simulink model "SF006A_TEstimn"  (R2013b)
settings: Solver=FixedStepDiscrete  StartTime=0.0  StopTime=1  FixedStep=0.1  RelTol=1e-3
values from neighbouring files (symbols this model uses):
  ARCHGLBPRM_100MILLISEC_SEC_F32 = DataDict.Constant    [SF006A_TEstimn_DataDict.m]
  ARCHGLBPRM_2MILLISEC_SEC_F32 = DataDict.Constant    [SF006A_TEstimn_DataDict.m]
  TEstimnAmbPwrMplr = DataDict.Calibration    [SF006A_TEstimn_DataDict.m]
  TEstimnAmbTSca = DataDict.Calibration    [SF006A_TEstimn_DataDict.m]
  TEstimnAssiMechAmbMplr = DataDict.Calibration    [SF006A_TEstimn_DataDict.m]
  TEstimnAssiMechCorrLim = DataDict.Calibration    [SF006A_TEstimn_DataDict.m]
  TEstimnAssiMechDampgSca = DataDict.Calibration    [SF006A_TEstimn_DataDict.m]
  TEstimnAssiMechDftT = DataDict.Calibration    [SF006A_TEstimn_DataDict.m]
  TEstimnAssiMechLLFilCoeffA1 = DataDict.Calibration    [SF006A_TEstimn_DataDict.m]
  TEstimnAssiMechLLFilCoeffB0 = DataDict.Calibration    [SF006A_TEstimn_DataDict.m]
  TEstimnAssiMechLLFilCoeffB1 = DataDict.Calibration    [SF006A_TEstimn_DataDict.m]
  TEstimnAssiMechSlew = DataDict.Calibration    [SF006A_TEstimn_DataDict.m]
  TESTIMNASSIMECHTHILIM_DEGCGRD_F32 = DataDict.Constant    [SF006A_TEstimn_DataDict.m]
  TESTIMNASSIMECHTLOLIM_DEGCGRD_F32 = DataDict.Constant    [SF006A_TEstimn_DataDict.m]
  TEstimnCorrnTAssiMech = DataDict.Calibration    [SF006A_TEstimn_DataDict.m]
  TEstimnCorrnTCu = DataDict.Calibration    [SF006A_TEstimn_DataDict.m]
  TEstimnCorrnTMag = DataDict.Calibration    [SF006A_TEstimn_DataDict.m]
  TEstimnCorrnTSi = DataDict.Calibration    [SF006A_TEstimn_DataDict.m]
  TEstimnCuAmbMplr = DataDict.Calibration    [SF006A_TEstimn_DataDict.m]
  TEstimnCuCorrnLim = DataDict.Calibration    [SF006A_TEstimn_DataDict.m]
  TEstimnCuLLFilCoeffA1 = DataDict.Calibration    [SF006A_TEstimn_DataDict.m]
  TEstimnCuLLFilCoeffB0 = DataDict.Calibration    [SF006A_TEstimn_DataDict.m]
  TEstimnCuLLFilCoeffB1 = DataDict.Calibration    [SF006A_TEstimn_DataDict.m]
  TEstimnEngTSca = DataDict.Calibration    [SF006A_TEstimn_DataDict.m]
  TESTIMNFETTHILIM_DEGCGRD_F32 = DataDict.Constant    [SF006A_TEstimn_DataDict.m]
  TESTIMNFETTLOLIM_DEGCGRD_F32 = DataDict.Constant    [SF006A_TEstimn_DataDict.m]
  TEstimnMagAmbMplr = DataDict.Calibration    [SF006A_TEstimn_DataDict.m]
  TEstimnMagCorrnLim = DataDict.Calibration    [SF006A_TEstimn_DataDict.m]
  TEstimnMagLLFilCoeffA1 = DataDict.Calibration    [SF006A_TEstimn_DataDict.m]
  TEstimnMagLLFilCoeffB0 = DataDict.Calibration    [SF006A_TEstimn_DataDict.m]
  TEstimnMagLLFilCoeffB1 = DataDict.Calibration    [SF006A_TEstimn_DataDict.m]
  TESTIMNMAGTHILIM_DEGCGRD_F32 = DataDict.Constant    [SF006A_TEstimn_DataDict.m]
  TESTIMNMAGTLOLIM_DEGCGRD_F32 = DataDict.Constant    [SF006A_TEstimn_DataDict.m]
  TEstimnSiAmbMplr = DataDict.Calibration    [SF006A_TEstimn_DataDict.m]
  TEstimnSiCorrnLim = DataDict.Calibration    [SF006A_TEstimn_DataDict.m]
  TEstimnSiLLFilCoeffA1 = DataDict.Calibration    [SF006A_TEstimn_DataDict.m]
  TEstimnSiLLFilCoeffB0 = DataDict.Calibration    [SF006A_TEstimn_DataDict.m]
  TEstimnSiLLFilCoeffB1 = DataDict.Calibration    [SF006A_TEstimn_DataDict.m]
  TEstimnWghtAvrgTDi = DataDict.Calibration    [SF006A_TEstimn_DataDict.m]
  TESTIMNWIDGTHILIM_DEGCGRD_F32 = DataDict.Constant    [SF006A_TEstimn_DataDict.m]
  TESTIMNWIDGTLOLIM_DEGCGRD_F32 = DataDict.Constant    [SF006A_TEstimn_DataDict.m]
undefined symbols (not defined in the file or in its folder): sigbuilder_block
libraries: NxtrLim x13, Fil x8, simulink x2
(part 1 of 3)
settings Model: Creator=PallavG  LastModifiedBy=FZG88Y
settings DataIOCC: LimitDataPoints=off  SaveFormat=Structure  ReturnWorkspaceOutputs=on
settings OptimizationCC: BlockReduction=off  InlineParams=on  ZeroExternalMemoryAtStartup=off  ZeroInternalMemoryAtStartup=off  OptimizeModelRefInitCode=on  LifeSpan=1
settings DebuggingCC: SignalInfNanChecking=error  SignalRangeChecking=warning  UnderspecifiedInitializationDetection=Simplified  SolverPrmCheckMsg=error  InheritedTsInSrcMsg=error  DiscreteInheritContinuousMsg=error  SingleTaskRateTransMsg=error  TasksWithSamePriorityMsg=error  SigSpecEnsureSampleTimeMsg=error  CheckMatrixSingularityMsg=error  IntegerOverflowMsg=error  ParameterUnderflowMsg=error  ParameterPrecisionLossMsg=error  ParameterTunabilityLossMsg=error  FixptConstUnderflowMsg=warning  FixptConstOverflowMsg=warning  VectorMatrixConversionMsg=error  SignalLabelMismatchMsg=error  UnconnectedInputMsg=error  UnconnectedOutputMsg=error  UnconnectedLineMsg=error  SFcnCompatibilityMsg=error  UniqueDataStoreMsg=warning  BusObjectLabelMismatch=error  RootOutportRequireBusObject=error  AssertControl=DisableAll  ModelReferenceIOMsg=error  ModelReferenceVersionMismatchMessage=warning  ModelReferenceIOMismatchMessage=error  ModelReferenceCSMismatchMessage=warning  ModelReferenceDataLoggingMessage=error  StateNameClashWarn=warning  StrictBusMsg=ErrorOnBusTreatedAsVector  NonBusSignalsTreatedAsBus=error  SFUnexpectedBacktrackingDiag=error  SFInvalidInputDataAccessInChartInitDiag=error  SFNoUnconditionalDefaultTransitionDiag=error  SFTransitionOutsideNaturalParentDiag=error  SFUnconditionalTransitionShadowingDiag=error  SFUndirectedBroadcastEventsDiag=error
settings ModelReferenceCC: ModelReferenceNumInstancesAllowed=Single
settings RTWCC: SystemTargetFile=autosar.tlc  GenCodeOnly=on  TemplateMakefile=ert_default_tmf  Description=AUTOSAR  GenerateReport=on  ProcessScript=autosar_make_rtw_hook  LaunchReport=on
settings CodeAppCC: GenerateComments=off  IgnoreCustomStorageClasses=off  CustomSymbolStrType=$N$R$M  CustomSymbolStrBlkIO=$N$M  SimulinkBlockComments=off
settings STFCustomTargetCC: ParMdlRefBuildCompliant=on  CompOptLevelCompliant=on  IncludeMdlTerminateFcn=off  CombineOutputUpdateFcns=on  SuppressErrorStatus=on  ERTFirstTimeCompliant=on  ERTCustomFileBanners=on  SupportNonFinite=off  SupportComplex=off  SupportContinuousTime=off  SupportNonInlinedSFcns=off  MATLABClassNameForMDSCustomization=Simulink.SoftwareTarget.ERTCustomization  AutosarCompliant=on  GRTInterface=off  SystemTargetFile=autosar.tlc
settings ERTTargetCC: CodeReplacementLibrary=ANSI_C  ConcurrentExecutionCompliant=off  IncludeMdlTerminateFcn=off  SuppressErrorStatus=on  SupportNonFinite=off  SupportComplex=off  ModelStepFunctionPrototypeControlCompliant=off  CPPClassGenCompliant=off  AutosarCompliant=on  InlinedParameterPlacement=NonHierarchical  ERTCustomFileTemplate=example_file_process.tlc  EnableUserReplacementTypes=on

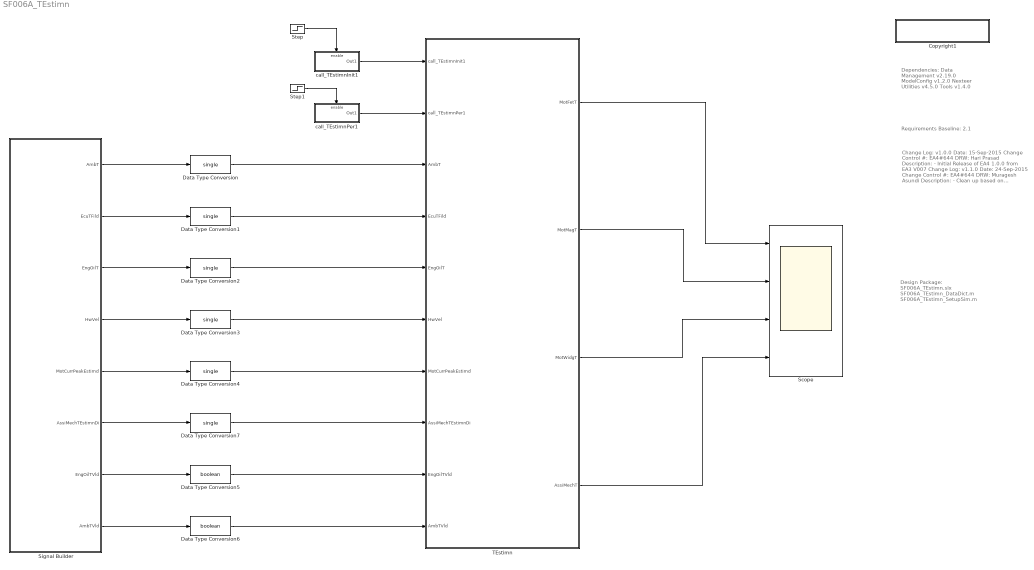
== system SF006A_TEstimn ==
  note: Requirements Baseline: 2.1
  note: Design Package:
      | SF006A_TEstimn.slx
      | SF006A_TEstimn_DataDict.m
      | SF006A_TEstimn_SetupSim.m
  note: Change Log:  v1.0.0
      | Date: 15-Sep-2015
      | Change Control #: EA4#644
      | DRW:  Hari Prasad
      | Description:
      | - Initial Release of EA4 1.0.0 from EA3 V007
      |
      | Change Log:  v1.1.0
      | Date: 24-Sep-2015
      | Change Control #: EA4#644
      | DRW:  Muragesh Asundi
      | Description:
      | - Clean up based on comments from SW team
  note: Dependencies:
      |    Data Management v2.19.0
      |    ModelConfig v1.2.0
      |    Nexteer Utilities v4.5.0
      |    Tools v1.4.0
  Copyright1 : Subsystem  Description=|  RequirementInfo={} %GIDa_31a5e494_f362_4315_ad68_df9135c8582b  mask(Copyright Information){none=on}
      | Copyright info block.                                               
      |                                                                     
      | Place copyright information at the top of every subsystem in design.
      mask prompts: none "No parameters"
      mask help: Place copyright information at the top of every subsystem in design.
      mask Display:
      | NxtrConf = 'Nexteer Confidential';
      | 
      | sys = bdroot; %handle for the current model ("system")
      | first = get_param(sys,'Created');
      | if(isempty(first))
      |     first = datestr(now,'yyyy');
      | else
      |     first = first(end-3:end);  %year is last four digits
      | end
      | 
      | last = get_param(sys,'LastModifiedDate');
      | if isempty(last)
      |     last = datestr(now,'yyyy');
      | else
      |     last = last(end-3:end);
      | end
      | 
      | if strcmp(first,last)
      |     fprintf('%s\nCopyright  %s Nexteer',NxtrConf,first);
      | else
      |     fprintf('%s\n%s%s-%s Nexteer',NxtrConf,char(169),first,last);
      | end
  Data Type Conversion{,1..4,7} (6 alike) : DataTypeConversion  OutDataTypeStr=single
  Data Type Conversion5 : DataTypeConversion  OutDataTypeStr=boolean
  Data Type Conversion6 : DataTypeConversion  OutDataTypeStr=boolean
  Scope : Scope  NumInputPorts=4
      settings: YMin=-5~-5~-5~-5  YMax=5~5~5~5
  Signal Builder : Subsystem  Tag=STV Subsys  LoadFcn=sigbuilder_block('load');  StartFcn=sigbuilder_block('start');  StopFcn=sigbuilder_block('stop');  ClipboardFcn=sigbuilder_block('clipboard');  mask(Sigbuilder block){}
      mask help: Simulink:masks:SigbuilderBlock_MD
      mask init:
      | if ~strcmp(get_param(bdroot(gcbh),'SimulationStatus'),'stopped') tuvar = sigbuilder_block('maskInit'); end
      settings: CopyFcn=sigbuilder_block('copy');  DeleteFcn=sigbuilder_block('delete');  ModelCloseFcn=sigbuilder_block('modelClose');  PreSaveFcn=sigbuilder_block('preSave');  PauseFcn=sigbuilder_block('pause');  ContinueFcn=sigbuilder_block('continue');  NameChangeFcn=sigbuilder_block('namechange');  OpenFcn=sigbuilder_block('open',[84 66 786.75 394.5 ]);  CloseFcn=sigbuilder_block('close');
      mask Display: plot(0, 0, 100, 100,[2, 2, 32, 32, 2], [68, 8, 8, 68, 68],[32, 2], [38, 38], [32, 19, 2],[53, 60, 44], [32, 17, 17, 2],[16, 16, 31, 31]);txt = getActiveGroup(gcbh);text(2, 100, txt,'verticalAlignment', 'top');
  Step : Step  Time=.001  Before=1  After=0  SampleTime=0
  Step1 : Step  Time=0.001  SampleTime=0.1
  TEstimn : Subsystem  RequirementInfo={'linktype_rmi_doors' '0000a528 (/E-STEER Core/SubSystem Specifications/Application Functions/SF006A Temperature Estimation)' '#SF006A_113' 'true' 'REQ: SF006A_113' '' } %GIDa_45cdad98_892c_499b_8f4d_04ff41f4306a
  call_TEstimnInit1 : Subsystem  TreatAsAtomicUnit=on
  call_TEstimnPer1 : Subsystem  TreatAsAtomicUnit=on
  wires:
  TEstimn/4(AssiMechT) -> Scope/4
  TEstimn/3(MotWidgT) -> Scope/3
  TEstimn/2(MotMagT) -> Scope/2
  TEstimn/1(MotFetT) -> Scope/1
  Data Type Conversion/1 -> TEstimn/3(AmbT)
  Data Type Conversion1/1 -> TEstimn/4(EcuTFild)
  Data Type Conversion2/1 -> TEstimn/5(EngOilT)
  Data Type Conversion3/1 -> TEstimn/6(HwVel)
  Data Type Conversion4/1 -> TEstimn/7(MotCurrPeakEstimd)
  Data Type Conversion7/1 -> TEstimn/8(AssiMechTEstimnDi)
  Signal Builder/7(EngOilTVld) -> Data Type Conversion5/1
  Signal Builder/2(EcuTFild) -> Data Type Conversion1/1
  Signal Builder/5(MotCurrPeakEstimd) -> Data Type Conversion4/1
  Signal Builder/3(EngOilT) -> Data Type Conversion2/1
  Signal Builder/6(AssiMechTEstimnDi) -> Data Type Conversion7/1
  Signal Builder/4(HwVel) -> Data Type Conversion3/1
  Signal Builder/1(AmbT) -> Data Type Conversion/1
  Data Type Conversion6/1 -> TEstimn/10(AmbTVld)
  Data Type Conversion5/1 -> TEstimn/9(EngOilTVld)
  Signal Builder/8(AmbTVld) -> Data Type Conversion6/1
  Step/1 -> call_TEstimnInit1/Enable
  call_TEstimnInit1/1(Out1) -> TEstimn/1(call_TEstimnInit1)
  Step1/1 -> call_TEstimnPer1/Enable
  call_TEstimnPer1/1(Out1) -> TEstimn/2(call_TEstimnPer1)

== system SF006A_TEstimn/Copyright1 ==

== system SF006A_TEstimn/Signal Builder ==
  Demux : Demux  Tag=STV Demux  Outputs=8
  FromWs : FromWorkspace  Tag=STV FromWs  VariableName=tuvar  SampleTime=0
      SigBuilderData=|
      | common.afterFinalStr = 'Extrapolate'
      | common.sampleTime = 0
      | dataSet(1).timeRange = [0 0.11]
      | dataSet(1).name = 'TestCase1'
      | dataSet(2).timeRange = [0 0.11]
      | dataSet(2).name = 'TestCase2'
      | dataSet(3).timeRange = [0 0.11]
      | dataSet(3).name = 'TestCase3'
      | dataSet(4).timeRange = [0 0.11]
      | dataSet(4).name = 'TestCase4'
      | dataSet(5).timeRange = [0 0.11]
      | dataSet(5).name = 'TestCase5'
      | dataSet(6).timeRange = [0 0.11]
      | dataSet(6).name = 'TestCase6'
      | sbobj.Name = 'Signal Builder'
      | sbobj.Groups(1).Name = 'TestCase1'
      | sbobj.Groups(1).Signals(1).Name = 'AmbT'
      | sbobj.Groups(1).Signals(1).XData = [0 0.002 0.004 0.006 0.008 0.01 0.012 0.014 0.016 0.018 0.02 0.022 0.024 0.026 0.028 0.03 0.032 0.034 0.036 0.038 0.04 0.042 0.044 0.046 0.048 0.05 0.052 0.054 0.056 0.058 0.06 0.062 0.064 0.066 0.068 0.07 0.072 0.074 0.076 0.078 0.08 0.082 0.084 0.086 0.088 0.09 0.092 0.094 0.096 0.098 0.1 0.102 0.104 0.106 0.108 0.11]
      | sbobj.Groups(1).Signals(1).YData = [0 0 0 0 0 0 0 0 0 0 0 0 0 0 0 0 0 0 0 0 0 0 0 0 0 0 0 0 0 0 0 0 0 0 0 0 0 0 0 0 0 0 0 0 0 0 0 0 0 0 0 0 0 0 0 0]
      | sbobj.Groups(1).Signals(2).Name = 'EcuTFild'
      | sbobj.Groups(1).Signals(2).XData = [0 0.002 0.004 0.006 0.008 0.01 0.012 0.014 0.016 0.018 0.02 0.022 0.024 0.026 0.028 0.03 0.032 0.034 0.036 0.038 0.04 0.042 0.044 0.046 0.048 0.05 0.052 0.054 0.056 0.058 0.06 0.062 0.064 0.066 0.068 0.07 0.072 0.074 0.076 0.078 0.08 0.082 0.084 0.086 0.088 0.09 0.092 0.094 0.096 0.098 0.1 0.102 0.104 0.106 0.108 0.11]
      | sbobj.Groups(1).Signals(2).YData = [50 50 23 -10 50 -3 50 50 -50 50 50 -25 50 50 -18 50 50 100 50 34 50 67 50 50 50 123 50 50 50 88 50 111 50 50 50 92 50 50 146 50 50 50 50 50 50 50 50 50 50 50 50 50 50 50 50 50]
      | sbobj.Groups(1).Signals(3).Name = 'EngOilT'
      | sbobj.Groups(1).Signals(3).XData = [0 0.002 0.004 0.006 0.008 0.01 0.012 0.014 0.016 0.018 0.02 0.022 0.024 0.026 0.028 0.03 0.032 0.034 0.036 0.038 0.04 0.042 0.044 0.046 0.048 0.05 0.052 0.054 0.056 0.058 0.06 0.062 0.064 0.066 0.068 0.07 0.072 0.074 0.076 0.078 0.08 0.082 0.084 0.086 0.088 0.09 0.092 0.094 0.096 0.098 0.1 0.102 0.104 0.106 0.108 0.11]
      | sbobj.Groups(1).Signals(3).YData = [5 5 5 5 5 5 5 5 5 5 5 5 5 5 -5 5 5 5 5 -20 5 5 5 5 -10 5 5 5 5 5 5 5 5 5 5 5 5 5 5 5 5 5 5 5 5 5 5 5 5 5 5 5 5 5 5 5]
      | sbobj.Groups(1).Signals(4).Name = 'HwVel'
      | sbobj.Groups(1).Signals(4).XData = [0 0.002 0.004 0.006 0.008 0.01 0.012 0.014 0.016 0.018 0.02 0.022 0.024 0.026 0.028 0.03 0.032 0.034 0.036 0.038 0.04 0.042 0.044 0.046 0.048 0.05 0.052 0.054 0.056 0.058 0.06 0.062 0.064 0.066 0.068 0.07 0.072 0.074 0.076 0.078 0.08 0.082 0.084 0.086 0.088 0.09 0.092 0.094 0.096 0.098 0.1 0.102 0.104 0.106 0.108 0.11]
      | sbobj.Groups(1).Signals(4).YData = [3 3 3 3 3 3 3 3 3 3 3 3 3 3 3 3 3 3 3 3 3 3 3 3 3 3 3 3 3 3 3 3 3 3 3 3 3 3 3 3 3 3 3 3 3 3 3 3 3 3 3 3 3 3 3 3]
      | sbobj.Groups(1).Signals(5).Name = 'MotCurrPeakEstimd'
      | sbobj.Groups(1).Signals(5).XData = [0 0.002 0.004 0.006 0.008 0.01 0.012 0.014 0.016 0.018 0.02 0.022 0.024 0.026 0.028 0.03 0.032 0.034 0.036 0.038 0.04 0.042 0.044 0.046 0.048 0.05 0.052 0.054 0.056 0.058 0.06 0.062 0.064 0.066 0.068 0.07 0.072 0.074 0.076 0.078 0.08 0.082 0.084 0.086 0.088 0.09 0.092 0.094 0.096 0.098 0.1 0.102 0.104 0.106 0.108 0.11]
      | sbobj.Groups(1).Signals(5).YData = [5 5 5 5 5 5 5 5 5 5 5 5 5 5 5 5 5 5 5 5 5 5 5 5 5 5 5 5 5 5 5 5 5 5 5 5 5 5 5 5 5 5 5 5 5 5 5 5 5 5 5 5 5 5 5 5]
      | sbobj.Groups(1).Signals(6).Name = 'AssiMechTEstimnDi'
      | sbobj.Groups(1).Signals(6).XData = [0 0.002 0.004 0.006 0.008 0.01 0.012 0.014 0.016 0.018 0.02 0.022 0.024 0.026 0.028 0.03 0.032 0.034 0.036 0.038 0.04 0.042 0.044 0.046 0.048 0.05 0.052 0.054 0.056 0.058 0.06 0.062 0.064 0.066 0.068 0.07 0.072 0.074 0.076 0.078 0.08 0.082 0.084 0.086 0.088 0.09 0.092 0.094 0.096 0.098 0.1 0.102 0.104 0.106 0.108 0.11]
      | sbobj.Groups(1).Signals(6).YData = [0 0 0 0 0 0 0 0 0 0 0 0 0 0 0 0 0 0 0 0 0 0 0 0 0 0 0 0 0 0 0 0 0 0 0 0 0 0 0 0 0 0 0 0 0 0 0 0 0 0 0 0 0 0 0 0]
      | sbobj.Groups(1).Signals(7).Name = 'EngOilTVld'
      | sbobj.Groups(1).Signals(7).XData = [0 0.002 0.004 0.006 0.008 0.01 0.012 0.014 0.016 0.018 0.02 0.022 0.024 0.026 0.028 0.03 0.032 0.034 0.036 0.038 0.04 0.042 0.044 0.046 0.048 0.05 0.052 0.054 0.056 0.058 0.06 0.062 0.064 0.066 0.068 0.07 0.072 0.074 0.076 0.078 0.08 0.082 0.084 0.086 0.088 0.09 0.092 0.094 0.096 0.098 0.1 0.102 0.104 0.106 0.108 0.11]
      | sbobj.Groups(1).Signals(7).YData = [1 1 1 1 1 1 1 1 1 1 1 1 1 1 1 1 1 1 1 1 1 1 1 1 1 1 1 1 1 1 1 1 1 1 1 1 1 1 1 1 1 1 1 1 1 1 1 1 1 1 1 1 1 1 1 1]
      | sbobj.Groups(1).Signals(8).Name = 'AmbTVld'
      | sbobj.Groups(1).Signals(8).XData = [0 0.002 0.004 0.006 0.008 0.01 0.012 0.014 0.016 0.018 0.02 0.022 0.024 0.026 0.028 0.03 0.032 0.034 0.036 0.038 0.04 0.042 0.044 0.046 0.048 0.05 0.052 0.054 0.056 0.058 0.06 0.062 0.064 0.066 0.068 0.07 0.072 0.074 0.076 0.078 0.08 0.082 0.084 0.086 0.088 0.09 0.092 0.094 0.096 0.098 0.1 0.102 0.104 0.106 0.108 0.11]
      | sbobj.Groups(1).Signals(8).YData = [1 1 1 1 1 1 1 1 1 1 1 1 1 1 1 1 1 1 1 1 1 1 1 1 1 1 1 1 1 1 1 1 1 1 1 1 1 1 1 1 1 1 1 1 1 1 1 1 1 1 1 1 1 1 1 1]
      | sbobj.Groups(1).TimeRange = [0 0.11]
      | sbobj.Groups(2).Name = 'TestCase2'
      | sbobj.Groups(2).Signals(1).Name = 'AmbT'
      | sbobj.Groups(2).Signals(1).XData = [0 0.002 0.004 0.006 0.008 0.01 0.012 0.014 0.016 0.018 0.02 0.022 0.024 0.026 0.028 0.03 0.032 0.034 0.036 0.038 0.04 0.042 0.044 0.046 0.048 0.05 0.052 0.054 0.056 0.058 0.06 0.062 0.064 0.066 0.068 0.07 0.072 0.074 0.076 0.078 0.08 0.082 0.084 0.086 0.088 0.09 0.092 0.094 0.096 0.098 0.1 0.102 0.104 0.106 0.108 0.11]
      | sbobj.Groups(2).Signals(1).YData = [0 0 0 0 0 0 0 0 0 0 0 0 0 0 0 0 0 0 0 0 0 0 0 0 0 0 0 0 0 0 0 0 0 0 0 0 0 0 0 0 0 0 0 0 0 0 0 0 0 0 0 0 0 0 0 0]
      | sbobj.Groups(2).Signals(2).Name = 'EcuTFild'
      | sbobj.Groups(2).Signals(2).XData = [0 0.002 0.004 0.006 0.008 0.01 0.012 0.014 0.016 0.018 0.02 0.022 0.024 0.026 0.028 0.03 0.032 0.034 0.036 0.038 0.04 0.042 0.044 0.046 0.048 0.05 0.052 0.054 0.056 0.058 0.06 0.062 0.064 0.066 0.068 0.07 0.072 0.074 0.076 0.078 0.08 0.082 0.084 0.086 0.088 0.09 0.092 0.094 0.096 0.098 0.1 0.102 0.104 0.106 0.108 0.11]
      | sbobj.Groups(2).Signals(2).YData = [50 50 50 50 50 50 50 50 50 50 50 50 50 50 50 50 50 50 50 50 50 50 50 50 50 50 50 50 50 50 50 50 50 50 50 50 50 50 50 50 50 50 50 50 50 50 50 50 50 50 50 50 50 50 50 50]
      | sbobj.Groups(2).Signals(3).Name = 'EngOilT'
      | sbobj.Groups(2).Signals(3).XData = [0 0.002 0.004 0.006 0.008 0.01 0.012 0.014 0.016 0.018 0.02 0.022 0.024 0.026 0.028 0.03 0.032 0.034 0.036 0.038 0.04 0.042 0.044 0.046 0.048 0.05 0.052 0.054 0.056 0.058 0.06 0.062 0.064 0.066 0.068 0.07 0.072 0.074 0.076 0.078 0.08 0.082 0.084 0.086 0.088 0.09 0.092 0.094 0.096 0.098 0.1 0.102 0.104 0.106 0.108 0.11]
      | sbobj.Groups(2).Signals(3).YData = [-20 5 -11 5 5 -2 5 22 5 5 -8 5 98 5 -5 5 -50 5 5 -20 5 5 100 5 -10 5 59 5 5 67 5 5 5 90 5 -1 5 88 5 5 1 5 5 5 23 5 56 5 5 5 5 123 5 0 5 102]
      | sbobj.Groups(2).Signals(4).Name = 'HwVel'
      | sbobj.Groups(2).Signals(4).XData = [0 0.002 0.004 0.006 0.008 0.01 0.012 0.014 0.016 0.018 0.02 0.022 0.024 0.026 0.028 0.03 0.032 0.034 0.036 0.038 0.04 0.042 0.044 0.046 0.048 0.05 0.052 0.054 0.056 0.058 0.06 0.062 0.064 0.066 0.068 0.07 0.072 0.074 0.076 0.078 0.08 0.082 0.084 0.086 0.088 0.09 0.092 0.094 0.096 0.098 0.1 0.102 0.104 0.106 0.108 0.11]
      | sbobj.Groups(2).Signals(4).YData = [3 3 3 3 3 3 3 3 3 3 3 3 3 3 3 3 3 3 3 3 3 3 3 3 3 3 3 3 3 3 3 3 3 3 3 3 3 3 3 3 3 3 3 3 3 3 3 3 3 3 3 3 3 3 3 3]
      | sbobj.Groups(2).Signals(5).Name = 'MotCurrPeakEstimd'
      | sbobj.Groups(2).Signals(5).XData = [0 0.002 0.004 0.006 0.008 0.01 0.012 0.014 0.016 0.018 0.02 0.022 0.024 0.026 0.028 0.03 0.032 0.034 0.036 0.038 0.04 0.042 0.044 0.046 0.048 0.05 0.052 0.054 0.056 0.058 0.06 0.062 0.064 0.066 0.068 0.07 0.072 0.074 0.076 0.078 0.08 0.082 0.084 0.086 0.088 0.09 0.092 0.094 0.096 0.098 0.1 0.102 0.104 0.106 0.108 0.11]
      | sbobj.Groups(2).Signals(5).YData = [5 5 5 5 5 5 5 5 5 5 5 5 5 5 5 5 5 5 5 5 5 5 5 5 5 5 5 5 5 5 5 5 5 5 5 5 5 5 5 5 5 5 5 5 5 5 5 5 5 5 5 5 5 5 5 5]
      | sbobj.Groups(2).Signals(6).Name = 'AssiMechTEstimnDi'
      | sbobj.Groups(2).Signals(6).XData = [0 0.002 0.004 0.006 0.008 0.01 0.012 0.014 0.016 0.018 0.02 0.022 0.024 0.026 0.028 0.03 0.032 0.034 0.036 0.038 0.04 0.042 0.044 0.046 0.048 0.05 0.052 0.054 0.056 0.058 0.06 0.062 0.064 0.066 0.068 0.07 0.072 0.074 0.076 0.078 0.08 0.082 0.084 0.086 0.088 0.09 0.092 0.094 0.096 0.098 0.1 0.102 0.104 0.106 0.108 0.11]
      | sbobj.Groups(2).Signals(6).YData = [0 0 0 0 0 0 0 0 0 0 0 0 0 0 0 0 0 0 0 0 0 0 0 0 0 0 0 0 0 0 0 0 0 0 0 0 0 0 0 0 0 0 0 0 0 0 0 0 0 0 0 0 0 0 0 0]
      | sbobj.Groups(2).Signals(7).Name = 'EngOilTVld'
      | sbobj.Groups(2).Signals(7).XData = [0 0.002 0.004 0.006 0.008 0.01 0.012 0.014 0.016 0.018 0.02 0.022 0.024 0.026 0.028 0.03 0.032 0.034 0.036 0.038 0.04 0.042 0.044 0.046 0.048 0.05 0.052 0.054 0.056 0.058 0.06 0.062 0.064 0.066 0.068 0.07 0.072 0.074 0.076 0.078 0.08 0.082 0.084 0.086 0.088 0.09 0.092 0.094 0.096 0.098 0.1 0.102 0.104 0.106 0.108 0.11]
      | sbobj.Groups(2).Signals(7).YData = [1 1 1 1 1 1 1 1 1 1 1 1 1 1 1 1 1 1 1 1 1 1 1 1 1 1 1 1 1 1 1 1 1 1 1 1 1 1 1 1 1 1 1 1 1 1 1 1 1 1 1 1 1 1 1 1]
      | sbobj.Groups(2).Signals(8).Name = 'AmbTVld'
      | sbobj.Groups(2).Signals(8).XData = [0 0.002 0.004 0.006 0.008 0.01 0.012 0.014 0.016 0.018 0.02 0.022 0.024 0.026 0.028 0.03 0.032 0.034 0.036 0.038 0.04 0.042 0.044 0.046 0.048 0.05 0.052 0.054 0.056 0.058 0.06 0.062 0.064 0.066 0.068 0.07 0.072 0.074 0.076 0.078 0.08 0.082 0.084 0.086 0.088 0.09 0.092 0.094 0.096 0.098 0.1 0.102 0.104 0.106 0.108 0.11]
      | sbobj.Groups(2).Signals(8).YData = [1 1 1 1 1 1 1 1 1 1 1 1 1 1 1 1 1 1 1 1 1 1 1 1 1 1 1 1 1 1 1 1 1 1 1 1 1 1 1 1 1 1 1 1 1 1 1 1 1 1 1 1 1 1 1 1]
      | sbobj.Groups(2).TimeRange = [0 0.11]
      | sbobj.Groups(3).Name = 'TestCase3'
      | sbobj.Groups(3).Signals(1).Name = 'AmbT'
      | sbobj.Groups(3).Signals(1).XData = [0 0.002 0.004 0.006 0.008 0.01 0.012 0.014 0.016 0.018 0.02 0.022 0.024 0.026 0.028 0.03 0.032 0.034 0.036 0.038 0.04 0.042 0.044 0.046 0.048 0.05 0.052 0.054 0.056 0.058 0.06 0.062 0.064 0.066 0.068 0.07 0.072 0.074 0.076 0.078 0.08 0.082 0.084 0.086 0.088 0.09 0.092 0.094 0.096 0.098 0.1 0.102 0.104 0.106 0.108 0.11]
      | sbobj.Groups(3).Signals(1).YData = [0 0 0 0 0 0 0 0 0 0 0 0 0 0 0 0 0 0 0 0 0 0 0 0 0 0 0 0 0 0 0 0 0 0 0 0 0 0 0 0 0 0 0 0 0 0 0 0 0 0 0 0 0 0 0 0]
      | sbobj.Groups(3).Signals(2).Name = 'EcuTFild'
      | sbobj.Groups(3).Signals(2).XData = [0 0.002 0.004 0.006 0.008 0.01 0.012 0.014 0.016 0.018 0.02 0.022 0.024 0.026 0.028 0.03 0.032 0.034 0.036 0.038 0.04 0.042 0.044 0.046 0.048 0.05 0.052 0.054 0.056 0.058 0.06 0.062 0.064 0.066 0.068 0.07 0.072 0.074 0.076 0.078 0.08 0.082 0.084 0.086 0.088 0.09 0.092 0.094 0.096 0.098 0.1 0.102 0.104 0.106 0.108 0.11]
      | sbobj.Groups(3).Signals(2).YData = [50 50 50 50 50 50 50 50 50 50 50 50 50 50 50 50 50 50 50 50 50 50 50 50 50 50 50 50 50 50 50 50 50 50 50 50 50 50 50 50 50 50 50 50 50 50 50 50 50 50 50 50 50 50 50 50]
      | sbobj.Groups(3).Signals(3).Name = 'EngOilT'
      | sbobj.Groups(3).Signals(3).XData = [0 0.002 0.004 0.006 0.008 0.01 0.012 0.014 0.016 0.018 0.02 0.022 0.024 0.026 0.028 0.03 0.032 0.034 0.036 0.038 0.04 0.042 0.044 0.046 0.048 0.05 0.052 0.054 0.056 0.058 0.06 0.062 0.064 0.066 0.068 0.07 0.072 0.074 0.076 0.078 0.08 0.082 0.084 0.086 0.088 0.09 0.092 0.094 0.096 0.098 0.1 0.102 0.104 0.106 0.108 0.11]
      | sbobj.Groups(3).Signals(3).YData = [5 5 5 5 5 5 5 5 5 5 5 5 5 5 -5 5 5 5 5 -20 5 5 5 5 -10 5 5 5 5 5 5 5 5 5 5 5 5 5 5 5 5 5 5 5 5 5 5 5 5 5 5 5 5 5 5 5]
      | sbobj.Groups(3).Signals(4).Name = 'HwVel'
      | sbobj.Groups(3).Signals(4).XData = [0 0.002 0.004 0.006 0.008 0.01 0.012 0.014 0.016 0.018 0.02 0.022 0.024 0.026 0.028 0.03 0.032 0.034 0.036 0.038 0.04 0.042 0.044 0.046 0.048 0.05 0.052 0.054 0.056 0.058 0.06 0.062 0.064 0.066 0.068 0.07 0.072 0.074 0.076 0.078 0.08 0.082 0.084 0.086 0.088 0.09 0.092 0.094 0.096 0.098 0.1 0.102 0.104 0.106 0.108 0.11]
      | sbobj.Groups(3).Signals(4).YData = [-42 -40 -30 32 3 3 3 33 3 40 3 3 3 3 23 3 3 0 3 3 3 3 29 3 3 10 3 3 3 -1 3 3 3 3 -3 3 3 3 3 18 3 3 -5 3 11 3 3 -10 3 3 9 3 3 40 21 42]
      | sbobj.Groups(3).Signals(5).Name = 'MotCurrPeakEstimd'
      | sbobj.Groups(3).Signals(5).XData = [0 0.002 0.004 0.006 0.008 0.01 0.012 0.014 0.016 0.018 0.02 0.022 0.024 0.026 0.028 0.03 0.032 0.034 0.036 0.038 0.04 0.042 0.044 0.046 0.048 0.05 0.052 0.054 0.056 0.058 0.06 0.062 0.064 0.066 0.068 0.07 0.072 0.074 0.076 0.078 0.08 0.082 0.084 0.086 0.088 0.09 0.092 0.094 0.096 0.098 0.1 0.102 0.104 0.106 0.108 0.11]
      | sbobj.Groups(3).Signals(5).YData = [5 5 5 5 5 5 5 5 5 5 5 5 5 5 5 5 5 5 5 5 5 5 5 5 5 5 5 5 5 5 5 5 5 5 5 5 5 5 5 5 5 5 5 5 5 5 5 5 5 5 5 5 5 5 5 5]
      | sbobj.Groups(3).Signals(6).Name = 'AssiMechTEstimnDi'
      | sbobj.Groups(3).Signals(6).XData = [0 0.002 0.004 0.006 0.008 0.01 0.012 0.014 0.016 0.018 0.02 0.022 0.024 0.026 0.028 0.03 0.032 0.034 0.036 0.038 0.04 0.042 0.044 0.046 0.048 0.05 0.052 0.054 0.056 0.058 0.06 0.062 0.064 0.066 0.068 0.07 0.072 0.074 0.076 0.078 0.08 0.082 0.084 0.086 0.088 0.09 0.092 0.094 0.096 0.098 0.1 0.102 0.104 0.106 0.108 0.11]
      | sbobj.Groups(3).Signals(6).YData = [0 0 0 0 0 0 0 0 0 0 0 0 0 0 0 0 0 0 0 0 0 0 0 0 0 0 0 0 0 0 0 0 0 0 0 0 0 0 0 0 0 0 0 0 0 0 0 0 0 0 0 0 0 0 0 0]
      | sbobj.Groups(3).Signals(7).Name = 'EngOilTVld'
      | sbobj.Groups(3).Signals(7).XData = [0 0.002 0.004 0.006 0.008 0.01 0.012 0.014 0.016 0.018 0.02 0.022 0.024 0.026 0.028 0.03 0.032 0.034 0.036 0.038 0.04 0.042 0.044 0.046 0.048 0.05 0.052 0.054 0.056 0.058 0.06 0.062 0.064 0.066 0.068 0.07 0.072 0.074 0.076 0.078 0.08 0.082 0.084 0.086 0.088 0.09 0.092 0.094 0.096 0.098 0.1 0.102 0.104 0.106 0.108 0.11]
      | sbobj.Groups(3).Signals(7).YData = [1 1 1 1 1 1 1 1 1 1 1 1 1 1 1 1 1 1 1 1 1 1 1 1 1 1 1 1 1 1 1 1 1 1 1 1 1 1 1 1 1 1 1 1 1 1 1 1 1 1 1 1 1 1 1 1]
      | sbobj.Groups(3).Signals(8).Name = 'AmbTVld'
      | sbobj.Groups(3).Signals(8).XData = [0 0.002 0.004 0.006 0.008 0.01 0.012 0.014 0.016 0.018 0.02 0.022 0.024 0.026 0.028 0.03 0.032 0.034 0.036 0.038 0.04 0.042 0.044 0.046 0.048 0.05 0.052 0.054 0.056 0.058 0.06 0.062 0.064 0.066 0.068 0.07 0.072 0.074 0.076 0.078 0.08 0.082 0.084 0.086 0.088 0.09 0.092 0.094 0.096 0.098 0.1 0.102 0.104 0.106 0.108 0.11]
      | sbobj.Groups(3).Signals(8).YData = [1 1 1 1 1 1 1 1 1 1 1 1 1 1 1 1 1 1 1 1 1 1 1 1 1 1 1 1 1 1 1 1 1 1 1 1 1 1 1 1 1 1 1 1 1 1 1 1 1 1 1 1 1 1 1 1]
      | sbobj.Groups(3).TimeRange = [0 0.11]
      | sbobj.Groups(4).Name = 'TestCase4'
      | sbobj.Groups(4).Signals(1).Name = 'AmbT'
      | sbobj.Groups(4).Signals(1).XData = [0 0.002 0.004 0.006 0.008 0.01 0.012 0.014 0.016 0.018 0.02 0.022 0.024 0.026 0.028 0.03 0.032 0.034 0.036 0.038 0.04 0.042 0.044 0.046 0.048 0.05 0.052 0.054 0.056 0.058 0.06 0.062 0.064 0.066 0.068 0.07 0.072 0.074 0.076 0.078 0.08 0.082 0.084 0.086 0.088 0.09 0.092 0.094 0.096 0.098 0.1 0.102 0.104 0.106 0.108 0.11]
      | sbobj.Groups(4).Signals(1).YData = [0 0 0 0 0 0 0 0 0 0 0 0 0 0 0 0 0 0 0 0 0 0 0 0 0 0 0 0 0 0 0 0 0 0 0 0 0 0 0 0 0 0 0 0 0 0 0 0 0 0 0 0 0 0 0 0]
      | sbobj.Groups(4).Signals(2).Name = 'EcuTFild'
      | sbobj.Groups(4).Signals(2).XData = [0 0.002 0.004 0.006 0.008 0.01 0.012 0.014 0.016 0.018 0.02 0.022 0.024 0.026 0.028 0.03 0.032 0.034 0.036 0.038 0.04 0.042 0.044 0.046 0.048 0.05 0.052 0.054 0.056 0.058 0.06 0.062 0.064 0.066 0.068 0.07 0.072 0.074 0.076 0.078 0.08 0.082 0.084 0.086 0.088 0.09 0.092 0.094 0.096 0.098 0.1 0.102 0.104 0.106 0.108 0.11]
      | sbobj.Groups(4).Signals(2).YData = [50 50 50 50 50 50 50 50 50 50 50 50 50 50 50 50 50 50 50 50 50 50 50 50 50 50 50 50 50 50 50 50 50 50 50 50 50 50 50 50 50 50 50 50 50 50 50 50 50 50 50 50 50 50 50 50]
      | sbobj.Groups(4).Signals(3).Name = 'EngOilT'
      | sbobj.Groups(4).Signals(3).XData = [0 0.002 0.004 0.006 0.008 0.01 0.012 0.014 0.016 0.018 0.02 0.022 0.024 0.026 0.028 0.03 0.032 0.034 0.036 0.038 0.04 0.042 0.044 0.046 0.048 0.05 0.052 0.054 0.056 0.058 0.06 0.062 0.064 0.066 0.068 0.07 0.072 0.074 0.076 0.078 0.08 0.082 0.084 0.086 0.088 0.09 0.092 0.094 0.096 0.098 0.1 0.102 0.104 0.106 0.108 0.11]
      | sbobj.Groups(4).Signals(3).YData = [5 5 5 5 5 5 5 5 5 5 5 5 5 5 -5 5 5 5 5 -20 5 5 5 5 -10 5 5 5 5 5 5 5 5 5 5 5 5 5 5 5 5 5 5 5 5 5 5 5 5 5 5 5 5 5 5 5]
      | sbobj.Groups(4).Signals(4).Name = 'HwVel'
      | sbobj.Groups(4).Signals(4).XData = [0 0.002 0.004 0.006 0.008 0.01 0.012 0.014 0.016 0.018 0.02 0.022 0.024 0.026 0.028 0.03 0.032 0.034 0.036 0.038 0.04 0.042 0.044 0.046 0.048 0.05 0.052 0.054 0.056 0.058 0.06 0.062 0.064 0.066 0.068 0.07 0.072 0.074 0.076 0.078 0.08 0.082 0.084 0.086 0.088 0.09 0.092 0.094 0.096 0.098 0.1 0.102 0.104 0.106 0.108 0.11]
      | sbobj.Groups(4).Signals(4).YData = [3 3 3 3 3 3 3 3 3 3 3 3 3 3 3 3 3 3 3 3 3 3 3 3 3 3 3 3 3 3 3 3 3 3 3 3 3 3 3 3 3 3 3 3 3 3 3 3 3 3 3 3 3 3 3 3]
      | sbobj.Groups(4).Signals(5).Name = 'MotCurrPeakEstimd'
      | sbobj.Groups(4).Signals(5).XData = [0 0.002 0.004 0.006 0.008 0.01 0.012 0.014 0.016 0.018 0.02 0.022 0.024 0.026 0.028 0.03 0.032 0.034 0.036 0.038 0.04 0.042 0.044 0.046 0.048 0.05 0.052 0.054 0.056 0.058 0.06 0.062 0.064 0.066 0.068 0.07 0.072 0.074 0.076 0.078 0.08 0.082 0.084 0.086 0.088 0.09 0.092 0.094 0.096 0.098 0.1 0.102 0.104 0.106 0.108 0.11]
      | sbobj.Groups(4).Signals(5).YData = [100 5 5 30000 5 5 5 24000 5 5 456 5 5 21 5 5 3245 5 22 5 5 0 5 5 999 5 5 5 1919 5 5 5 34 5 5 5657 5 5 10000 5 5 9879 5 5 62500 5 5 5 66 5 5 0 5 9 5 100]
      | sbobj.Groups(4).Signals(6).Name = 'AssiMechTEstimnDi'
      | sbobj.Groups(4).Signals(6).XData = [0 0.002 0.004 0.006 0.008 0.01 0.012 0.014 0.016 0.018 0.02 0.022 0.024 0.026 0.028 0.03 0.032 0.034 0.036 0.038 0.04 0.042 0.044 0.046 0.048 0.05 0.052 0.054 0.056 0.058 0.06 0.062 0.064 0.066 0.068 0.07 0.072 0.074 0.076 0.078 0.08 0.082 0.084 0.086 0.088 0.09 0.092 0.094 0.096 0.098 0.1 0.102 0.104 0.106 0.108 0.11]
      | sbobj.Groups(4).Signals(6).YData = [0 0 0 0 0 0 0 0 0 0 0 0 0 0 0 0 0 0 0 0 0 0 0 0 0 0 0 0 0 0 0 0 0 0 0 0 0 0 0 0 0 0 0 0 0 0 0 0 0 0 0 0 0 0 0 0]
      | sbobj.Groups(4).Signals(7).Name = 'EngOilTVld'
      | sbobj.Groups(4).Signals(7).XData = [0 0.002 0.004 0.006 0.008 0.01 0.012 0.014 0.016 0.018 0.02 0.022 0.024 0.026 0.028 0.03 0.032 0.034 0.036 0.038 0.04 0.042 0.044 0.046 0.048 0.05 0.052 0.054 0.056 0.058 0.06 0.062 0.064 0.066 0.068 0.07 0.072 0.074 0.076 0.078 0.08 0.082 0.084 0.086 0.088 0.09 0.092 0.094 0.096 0.098 0.1 0.102 0.104 0.106 0.108 0.11]
      | sbobj.Groups(4).Signals(7).YData = [1 1 1 1 1 1 1 1 1 1 1 1 1 1 1 1 1 1 1 1 1 1 1 1 1 1 1 1 1 1 1 1 1 1 1 1 1 1 1 1 1 1 1 1 1 1 1 1 1 1 1 1 1 1 1 1]
      | sbobj.Groups(4).Signals(8).Name = 'AmbTVld'
      | sbobj.Groups(4).Signals(8).XData = [0 0.002 0.004 0.006 0.008 0.01 0.012 0.014 0.016 0.018 0.02 0.022 0.024 0.026 0.028 0.03 0.032 0.034 0.036 0.038 0.04 0.042 0.044 0.046 0.048 0.05 0.052 0.054 0.056 0.058 0.06 0.062 0.064 0.066 0.068 0.07 0.072 0.074 0.076 0.078 0.08 0.082 0.084 0.086 0.088 0.09 0.092 0.094 0.096 0.098 0.1 0.102 0.104 0.106 0.108 0.11]
      | sbobj.Groups(4).Signals(8).YData = [1 1 1 1 1 1 1 1 1 1 1 1 1 1 1 1 1 1 1 1 1 1 1 1 1 1 1 1 1 1 1 1 1 1 1 1 1 1 1 1 1 1 1 1 1 1 1 1 1 1 1 1 1 1 1 1]
      | sbobj.Groups(4).TimeRange = [0 0.11]
      | sbobj.Groups(5).Name = 'TestCase5'
      | sbobj.Groups(5).Signals(1).Name = 'AmbT'
      | sbobj.Groups(5).Signals(1).XData = [0 0.002 0.004 0.006 0.008 0.01 0.012 0.014 0.016 0.018 0.02 0.022 0.024 0.026 0.028 0.03 0.032 0.034 0.036 0.038 0.04 0.042 0.044 0.046 0.048 0.05 0.052 0.054 0.056 0.058 0.06 0.062 0.064 0.066 0.068 0.07 0.072 0.074 0.076 0.078 0.08 0.082 0.084 0.086 0.088 0.09 0.092 0.094 0.096 0.098 0.1 0.102 0.104 0.106 0.108 0.11]
      | sbobj.Groups(5).Signals(1).YData = [0 0 0 0 0 0 0 0 0 0 0 0 0 0 0 0 0 0 0 0 0 0 0 0 0 0 0 0 0 0 0 0 0 0 0 0 0 0 0 0 0 0 0 0 0 0 0 0 0 0 0 0 0 0 0 0]
      | sbobj.Groups(5).Signals(2).Name = 'EcuTFild'
      | sbobj.Groups(5).Signals(2).XData = [0 0.002 0.004 0.006 0.008 0.01 0.012 0.014 0.016 0.018 0.02 0.022 0.024 0.026 0.028 0.03 0.032 0.034 0.036 0.038 0.04 0.042 0.044 0.046 0.048 0.05 0.052 0.054 0.056 0.058 0.06 0.062 0.064 0.066 0.068 0.07 0.072 0.074 0.076 0.078 0.08 0.082 0.084 0.086 0.088 0.09 0.092 0.094 0.096 0.098 0.1 0.102 0.104 0.106 0.108 0.11]
      | sbobj.Groups(5).Signals(2).YData = [50 50 50 50 50 50 50 50 50 50 50 50 50 50 50 50 50 50 50 50 50 50 50 50 50 50 50 50 50 50 50 50 50 50 50 50 50 50 50 50 50 50 50 50 50 50 50 50 50 50 50 50 50 50 50 50]
      | sbobj.Groups(5).Signals(3).Name = 'EngOilT'
      | sbobj.Groups(5).Signals(3).XData = [0 0.002 0.004 0.006 0.008 0.01 0.012 0.014 0.016 0.018 0.02 0.022 0.024 0.026 0.028 0.03 0.032 0.034 0.036 0.038 0.04 0.042 0.044 0.046 0.048 0.05 0.052 0.054 0.056 0.058 0.06 0.062 0.064 0.066 0.068 0.07 0.072 0.074 0.076 0.078 0.08 0.082 0.084 0.086 0.088 0.09 0.092 0.094 0.096 0.098 0.1 0.102 0.104 0.106 0.108 0.11]
      | sbobj.Groups(5).Signals(3).YData = [5 5 5 5 5 5 5 5 5 5 5 5 5 5 -5 5 5 5 5 -20 5 5 5 5 -10 5 5 5 5 5 5 5 5 5 5 5 5 5 5 5 5 5 5 5 5 5 5 5 5 5 5 5 5 5 5 5]
      | sbobj.Groups(5).Signals(4).Name = 'HwVel'
      | sbobj.Groups(5).Signals(4).XData = [0 0.002 0.004 0.006 0.008 0.01 0.012 0.014 0.016 0.018 0.02 0.022 0.024 0.026 0.028 0.03 0.032 0.034 0.036 0.038 0.04 0.042 0.044 0.046 0.048 0.05 0.052 0.054 0.056 0.058 0.06 0.062 0.064 0.066 0.068 0.07 0.072 0.074 0.076 0.078 0.08 0.082 0.084 0.086 0.088 0.09 0.092 0.094 0.096 0.098 0.1 0.102 0.104 0.106 0.108 0.11]
      | sbobj.Groups(5).Signals(4).YData = [3 3 3 3 3 3 3 3 3 3 3 3 3 3 3 3 3 3 3 3 3 3 3 3 3 3 3 3 3 3 3 3 3 3 3 3 3 3 3 3 3 3 3 3 3 3 3 3 3 3 3 3 3 3 3 3]
      | sbobj.Groups(5).Signals(5).Name = 'MotCurrPeakEstimd'
      | sbobj.Groups(5).Signals(5).XData = [0 0.002 0.004 0.006 0.008 0.01 0.012 0.014 0.016 0.018 0.02 0.022 0.024 0.026 0.028 0.03 0.032 0.034 0.036 0.038 0.04 0.042 0.044 0.046 0.048 0.05 0.052 0.054 0.056 0.058 0.06 0.062 0.064 0.066 0.068 0.07 0.072 0.074 0.076 0.078 0.08 0.082 0.084 0.086 0.088 0.09 0.092 0.094 0.096 0.098 0.1 0.102 0.104 0.106 0.108 0.11]
      | sbobj.Groups(5).Signals(5).YData = [5 5 5 5 5 5 5 5 5 5 5 5 5 5 5 5 5 5 5 5 5 5 5 5 5 5 5 5 5 5 5 5 5 5 5 5 5 5 5 5 5 5 5 5 5 5 5 5 5 5 5 5 5 5 5 5]
      | sbobj.Groups(5).Signals(6).Name = 'AssiMechTEstimnDi'
      | sbobj.Groups(5).Signals(6).XData = [0 0.002 0.004 0.006 0.008 0.01 0.012 0.014 0.016 0.018 0.02 0.022 0.024 0.026 0.028 0.03 0.032 0.034 0.036 0.038 0.04 0.042 0.044 0.046 0.048 0.05 0.052 0.054 0.056 0.058 0.06 0.062 0.064 0.066 0.068 0.07 0.072 0.074 0.076 0.078 0.08 0.082 0.084 0.086 0.088 0.09 0.092 0.094 0.096 0.098 0.1 0.102 0.104 0.106 0.108 0.11]
      | sbobj.Groups(5).Signals(6).YData = [1 0 1 0 1 0 0 0 0 1 0 0 0 0 1 0 0 0 1 0 0 0 1 0 0 0 0 1 0 0 1 1 0 0 1 0 0 0 0 0 1 0 1 1 1 1 1 1 0 0 0 0 0 0 1 1]
      | sbobj.Groups(5).Signals(7).Name = 'EngOilTVld'
      | sbobj.Groups(5).Signals(7).XData = [0 0.002 0.004 0.006 0.008 0.01 0.012 0.014 0.016 0.018 0.02 0.022 0.024 0.026 0.028 0.03 0.032 0.034 0.036 0.038 0.04 0.042 0.044 0.046 0.048 0.05 0.052 0.054 0.056 0.058 0.06 0.062 0.064 0.066 0.068 0.07 0.072 0.074 0.076 0.078 0.08 0.082 0.084 0.086 0.088 0.09 0.092 0.094 0.096 0.098 0.1 0.102 0.104 0.106 0.108 0.11]
      | sbobj.Groups(5).Signals(7).YData = [1 1 1 1 1 1 1 1 1 1 1 1 1 1 1 1 1 1 1 1 1 1 1 1 1 1 1 1 1 1 1 1 1 1 1 1 1 1 1 1 1 1 1 1 1 1 1 1 1 1 1 1 1 1 1 1]
      | sbobj.Groups(5).Signals(8).Name = 'AmbTVld'
      | sbobj.Groups(5).Signals(8).XData = [0 0.002 0.004 0.006 0.008 0.01 0.012 0.014 0.016 0.018 0.02 0.022 0.024 0.026 0.028 0.03 0.032 0.034 0.036 0.038 0.04 0.042 0.044 0.046 0.048 0.05 0.052 0.054 0.056 0.058 0.06 0.062 0.064 0.066 0.068 0.07 0.072 0.074 0.076 0.078 0.08 0.082 0.084 0.086 0.088 0.09 0.092 0.094 0.096 0.098 0.1 0.102 0.104 0.106 0.108 0.11]
      | sbobj.Groups(5).Signals(8).YData = [1 1 1 1 1 1 1 1 1 1 1 1 1 1 1 1 1 1 1 1 1 1 1 1 1 1 1 1 1 1 1 1 1 1 1 1 1 1 1 1 1 1 1 1 1 1 1 1 1 1 1 1 1 1 1 1]
      | sbobj.Groups(5).TimeRange = [0 0.11]
      | sbobj.Groups(6).Name = 'TestCase6'
      | sbobj.Groups(6).Signals(1).Name = 'AmbT'
      | sbobj.Groups(6).Signals(1).XData = [0 0.002 0.004 0.006 0.008 0.01 0.012 0.014 0.016 0.018 0.02 0.022 0.024 0.026 0.028 0.03 0.032 0.034 0.036 0.038 0.04 0.042 0.044 0.046 0.048 0.05 0.052 0.054 0.056 0.058 0.06 0.062 0.064 0.066 0.068 0.07 0.072 0.074 0.076 0.078 0.08 0.082 0.084 0.086 0.088 0.09 0.092 0.094 0.096 0.098 0.1 0.102 0.104 0.106 0.108 0.11]
      | sbobj.Groups(6).Signals(1).YData = [0 0 0 0 0 0 0 0 0 0 0 0 0 0 0 0 0 0 0 0 0 0 0 0 0 0 0 0 0 0 0 0 0 0 0 0 0 0 0 0 0 0 0 0 0 0 0 0 0 0 0 0 0 0 0 0]
      | sbobj.Groups(6).Signals(2).Name = 'EcuTFild'
      | sbobj.Groups(6).Signals(2).XData = [0 0.002 0.004 0.006 0.008 0.01 0.012 0.014 0.016 0.018 0.02 0.022 0.024 0.026 0.028 0.03 0.032 0.034 0.036 0.038 0.04 0.042 0.044 0.046 0.048 0.05 0.052 0.054 0.056 0.058 0.06 0.062 0.064 0.066 0.068 0.07 0.072 0.074 0.076 0.078 0.08 0.082 0.084 0.086 0.088 0.09 0.092 0.094 0.096 0.098 0.1 0.102 0.104 0.106 0.108 0.11]
      | sbobj.Groups(6).Signals(2).YData = [50 50 50 50 50 50 50 50 50 50 50 50 50 50 50 50 50 50 50 50 50 50 50 50 50 50 50 50 50 50 50 50 50 50 50 50 50 50 50 50 50 50 50 50 50 50 50 50 50 50 50 50 50 50 50 50]
      | sbobj.Groups(6).Signals(3).Name = 'EngOilT'
      | sbobj.Groups(6).Signals(3).XData = [0 0.002 0.004 0.006 0.008 0.01 0.012 0.014 0.016 0.018 0.02 0.022 0.024 0.026 0.028 0.03 0.032 0.034 0.036 0.038 0.04 0.042 0.044 0.046 0.048 0.05 0.052 0.054 0.056 0.058 0.06 0.062 0.064 0.066 0.068 0.07 0.072 0.074 0.076 0.078 0.08 0.082 0.084 0.086 0.088 0.09 0.092 0.094 0.096 0.098 0.1 0.102 0.104 0.106 0.108 0.11]
      | sbobj.Groups(6).Signals(3).YData = [5 5 5 5 5 5 5 5 5 5 5 5 5 5 -5 5 5 5 5 -20 5 5 5 5 -10 5 5 5 5 5 5 5 5 5 5 5 5 5 5 5 5 5 5 5 5 5 5 5 5 5 5 5 5 5 5 5]
      | sbobj.Groups(6).Signals(4).Name = 'HwVel'
      | sbobj.Groups(6).Signals(4).XData = [0 0.002 0.004 0.006 0.008 0.01 0.012 0.014 0.016 0.018 0.02 0.022 0.024 0.026 0.028 0.03 0.032 0.034 0.036 0.038 0.04 0.042 0.044 0.046 0.048 0.05 0.052 0.054 0.056 0.058 0.06 0.062 0.064 0.066 0.068 0.07 0.072 0.074 0.076 0.078 0.08 0.082 0.084 0.086 0.088 0.09 0.092 0.094 0.096 0.098 0.1 0.102 0.104 0.106 0.108 0.11]
      | sbobj.Groups(6).Signals(4).YData = [3 3 3 3 3 3 3 3 3 3 3 3 3 3 3 3 3 3 3 3 3 3 3 3 3 3 3 3 3 3 3 3 3 3 3 3 3 3 3 3 3 3 3 3 3 3 3 3 3 3 3 3 3 3 3 3]
      | sbobj.Groups(6).Signals(5).Name = 'MotCurrPeakEstimd'
      | sbobj.Groups(6).Signals(5).XData = [0 0.002 0.004 0.006 0.008 0.01 0.012 0.014 0.016 0.018 0.02 0.022 0.024 0.026 0.028 0.03 0.032 0.034 0.036 0.038 0.04 0.042 0.044 0.046 0.048 0.05 0.052 0.054 0.056 0.058 0.06 0.062 0.064 0.066 0.068 0.07 0.072 0.074 0.076 0.078 0.08 0.082 0.084 0.086 0.088 0.09 0.092 0.094 0.096 0.098 0.1 0.102 0.104 0.106 0.108 0.11]
      | sbobj.Groups(6).Signals(5).YData = [5 5 5 5 5 5 5 5 5 5 5 5 5 5 5 5 5 5 5 5 5 5 5 5 5 5 5 5 5 5 5 5 5 5 5 5 5 5 5 5 5 5 5 5 5 5 5 5 5 5 5 5 5 5 5 5]
      | sbobj.Groups(6).Signals(6).Name = 'AssiMechTEstimnDi'
      | sbobj.Groups(6).Signals(6).XData = [0 0.002 0.004 0.006 0.008 0.01 0.012 0.014 0.016 0.018 0.02 0.022 0.024 0.026 0.028 0.03 0.032 0.034 0.036 0.038 0.04 0.042 0.044 0.046 0.048 0.05 0.052 0.054 0.056 0.058 0.06 0.062 0.064 0.066 0.068 0.07 0.072 0.074 0.076 0.078 0.08 0.082 0.084 0.086 0.088 0.09 0.092 0.094 0.096 0.098 0.1 0.102 0.104 0.106 0.108 0.11]
      | sbobj.Groups(6).Signals(6).YData = [1 0 1 0 1 0 0 0 0 1 0 0 0 0 1 0 0 0 1 0 0 1 1 1 0 0 0 1 0 0 1 1 1 1 1 1 1 1 0 0 1 0 1 1 1 1 1 1 0 0 0 0 1 1 1 1]
      | sbobj.Groups(6).Signals(7).Name = 'EngOilTVld'
      | sbobj.Groups(6).Signals(7).XData = [0 0.002 0.004 0.006 0.008 0.01 0.012 0.014 0.016 0.018 0.02 0.022 0.024 0.026 0.028 0.03 0.032 0.034 0.036 0.038 0.04 0.042 0.044 0.046 0.048 0.05 0.052 0.054 0.056 0.058 0.06 0.062 0.064 0.066 0.068 0.07 0.072 0.074 0.076 0.078 0.08 0.082 0.084 0.086 0.088 0.09 0.092 0.094 0.096 0.098 0.1 0.102 0.104 0.106 0.108 0.11]
      | sbobj.Groups(6).Signals(7).YData = [1 1 1 1 1 1 1 1 1 1 1 1 1 1 1 1 1 1 1 1 1 1 1 1 1 1 1 1 1 1 1 1 1 1 1 1 1 1 1 1 1 1 1 1 1 1 1 1 1 1 1 1 1 1 1 1]
      | sbobj.Groups(6).Signals(8).Name = 'AmbTVld'
      | sbobj.Groups(6).Signals(8).XData = [0 0.002 0.004 0.006 0.008 0.01 0.012 0.014 0.016 0.018 0.02 0.022 0.024 0.026 0.028 0.03 0.032 0.034 0.036 0.038 0.04 0.042 0.044 0.046 0.048 0.05 0.052 0.054 0.056 0.058 0.06 0.062 0.064 0.066 0.068 0.07 0.072 0.074 0.076 0.078 0.08 0.082 0.084 0.086 0.088 0.09 0.092 0.094 0.096 0.098 0.1 0.102 0.104 0.106 0.108 0.11]
      | sbobj.Groups(6).Signals(8).YData = [0 0 0 0 0 0 0 0 0 0 0 0 0 0 0 0 0 0 0 0 0 0 0 0 0 0 0 0 0 0 0 0 0 0 0 0 0 0 0 0 0 0 0 0 0 0 0 0 0 0 0 0 0 0 0 0]
      | sbobj.Groups(6).TimeRange = [0 0.11]
  AmbT : Outport
  EcuTFild : Outport  Tag=STV Outport  Port=2
  EngOilT : Outport  Tag=STV Outport  Port=3
  HwVel : Outport  Tag=STV Outport  Port=4
  MotCurrPeakEstimd : Outport  Tag=STV Outport  Port=5
  AssiMechTEstimnDi : Outport  Tag=STV Outport  Port=6
  EngOilTVld : Outport  Tag=STV Outport  Port=7
  AmbTVld : Outport  Tag=STV Outport  Port=8
  wires:
  Demux/1 -> AmbT/1
  FromWs/1 -> Demux/1
  Demux/2 -> EcuTFild/1
  Demux/3 -> EngOilT/1
  Demux/4 -> HwVel/1
  Demux/5 -> MotCurrPeakEstimd/1
  Demux/6 -> AssiMechTEstimnDi/1
  Demux/7 -> EngOilTVld/1
  Demux/8 -> AmbTVld/1

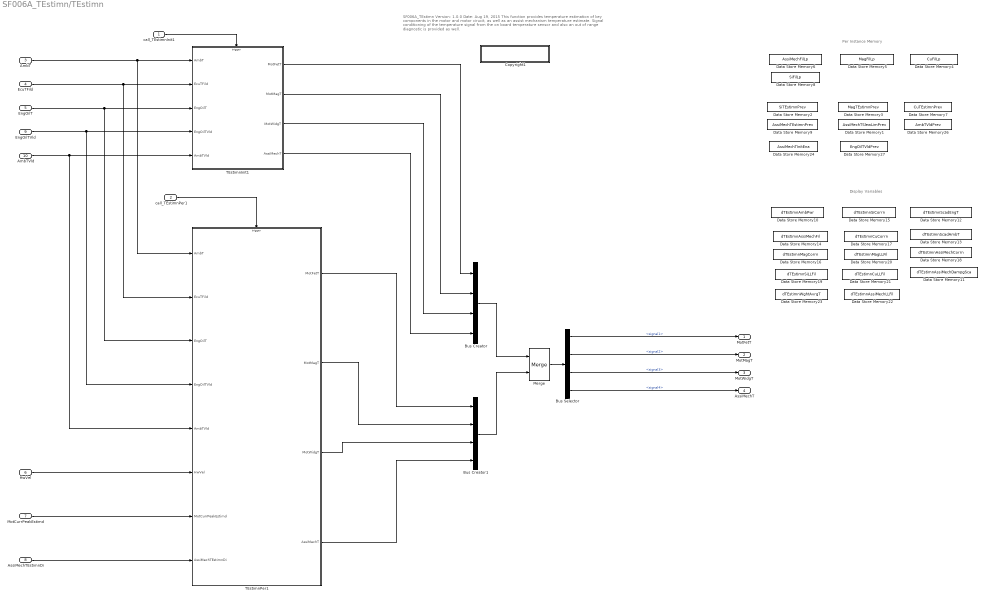
== system SF006A_TEstimn/TEstimn ==
  note: Per Instance Memory
  note: Display Variables
  note: SF006A_TEstimn       Version: 1.0.0                                                      Date:  Aug 19, 2015
      |
      | This function provides temperature estimation of key components in the motor and motor cirucit, as well as an assist mechanism temperature estimate.
      |  Signal conditioning of the temperature signal from the on board temperature sensor and also an out of range diagnostic is provided as well.
  call_TEstimnInit1 : Inport
  call_TEstimnPer1 : Inport  Port=2
  AmbT : Inport  RequirementInfo={'linktype_rmi_doors' '0000a528 (/E-STEER Core/SubSystem Specifications/Application Functions/SF006A Temperature Estimation)' '#SF006A_36' 'true' 'REQ: SF006A_36' '' } %GIDa_5d6b064d_6b6f_4541_a887_c0efbe9c0c94  Port=3
  EcuTFild : Inport  RequirementInfo={'linktype_rmi_doors' '0000a528 (/E-STEER Core/SubSystem Specifications/Application Functions/SF006A Temperature Estimation)' '#SF006A_169' 'true' 'REQ: SF006A_169' '' } %GIDa_7589b720_6e4c_4e94_96af_7b6fe1e4d0db  Port=4
  EngOilT : Inport  RequirementInfo={'linktype_rmi_doors' '0000a528 (/E-STEER Core/SubSystem Specifications/Application Functions/SF006A Temperature Estimation)' '#SF006A_35' 'true' 'REQ: SF006A_35' '' } %GIDa_5c47e2cc_0424_4f9b_9e07_6d85924c893e  Port=5
  HwVel : Inport  RequirementInfo={'linktype_rmi_doors' '0000a528 (/E-STEER Core/SubSystem Specifications/Application Functions/SF006A Temperature Estimation)' '#SF006A_33' 'true' 'REQ: SF006A_33' '' } %GIDa_66961606_1485_4273_a568_ee274f5fd10b  Port=6
  MotCurrPeakEstimd : Inport  RequirementInfo={'linktype_rmi_doors' '0000a528 (/E-STEER Core/SubSystem Specifications/Application Functions/SF006A Temperature Estimation)' '#SF006A_34' 'true' 'REQ: SF006A_34' '' } %GIDa_9ffd1575_018e_4c04_9a89_090695dc7784  Port=7
  AssiMechTEstimnDi : Inport  RequirementInfo={'linktype_rmi_doors' '0000a528 (/E-STEER Core/SubSystem Specifications/Application Functions/SF006A Temperature Estimation)' '#SF006A_39' 'true' 'REQ: SF006A_39' '' } %GIDa_64c39ffe_14e6_405a_a806_1cae4ba36277  Port=8
  EngOilTVld : Inport  RequirementInfo={'linktype_rmi_doors' '0000a528 (/E-STEER Core/SubSystem Specifications/Application Functions/SF006A Temperature Estimation)' '#SF006A_37' 'true' 'REQ: SF006A_37' '' } %GIDa_7d7a5cea_4edb_4765_a58d_84344722e689  Port=9
  AmbTVld : Inport  RequirementInfo={'linktype_rmi_doors' '0000a528 (/E-STEER Core/SubSystem Specifications/Application Functions/SF006A Temperature Estimation)' '#SF006A_37' 'true' 'REQ: SF006A_37' '' } %GIDa_744f25b6_7177_4752_87bb_5589619ff46a  Port=10
  Bus Creator : BusCreator
  Bus Creator1 : BusCreator
  Bus Selector : BusSelector  OutputSignals=signal1,signal2,signal3,signal4
  Copyright1 : Subsystem  Description=|  RequirementInfo={} %GIDa_40b2bef5_baed_40e1_9760_ec08ea904b84  mask(Copyright Information){none=on}
      | Copyright info block.                                               
      |                                                                     
      | Place copyright information at the top of every subsystem in design.
      mask prompts: none "No parameters"
      mask help: Place copyright information at the top of every subsystem in design.
      mask Display:
      | NxtrConf = 'Nexteer Confidential';
      | 
      | sys = bdroot; %handle for the current model ("system")
      | first = get_param(sys,'Created');
      | if(isempty(first))
      |     first = datestr(now,'yyyy');
      | else
      |     first = first(end-3:end);  %year is last four digits
      | end
      | 
      | last = get_param(sys,'LastModifiedDate');
      | if isempty(last)
      |     last = datestr(now,'yyyy');
      | else
      |     last = last(end-3:end);
      | end
      | 
      | if strcmp(first,last)
      |     fprintf('%s\nCopyright  %s Nexteer',NxtrConf,first);
      | else
      |     fprintf('%s\n%s%s-%s Nexteer',NxtrConf,char(169),first,last);
      | end
  Data Store Memory1 : DataStoreMemory  DataStoreName=AssiMechTSlewLimPrev  StateMustResolveToSignalObject=on
      settings: LockScale=on
  Data Store Memory10 : DataStoreMemory  DataStoreName=dTEstimnAmbPwr  StateMustResolveToSignalObject=on
  Data Store Memory11 : DataStoreMemory  DataStoreName=dTEstimnAssiMechDampgSca  StateMustResolveToSignalObject=on
  Data Store Memory12 : DataStoreMemory  DataStoreName=dTEstimnScadEngT  StateMustResolveToSignalObject=on
  Data Store Memory13 : DataStoreMemory  DataStoreName=dTEstimnScadAmbT  StateMustResolveToSignalObject=on
  Data Store Memory14 : DataStoreMemory  DataStoreName=dTEstimnAssiMechFil  StateMustResolveToSignalObject=on
  Data Store Memory15 : DataStoreMemory  DataStoreName=dTEstimnSiCorrn  StateMustResolveToSignalObject=on
  Data Store Memory16 : DataStoreMemory  DataStoreName=dTEstimnMagCorrn  StateMustResolveToSignalObject=on
  Data Store Memory17 : DataStoreMemory  DataStoreName=dTEstimnCuCorrn  StateMustResolveToSignalObject=on
  Data Store Memory18 : DataStoreMemory  DataStoreName=dTEstimnAssiMechCorrn  StateMustResolveToSignalObject=on
  Data Store Memory19 : DataStoreMemory  DataStoreName=dTEstimnSiLLFil  StateMustResolveToSignalObject=on
  Data Store Memory2 : DataStoreMemory  DataStoreName=SiTEstimnPrev  StateMustResolveToSignalObject=on
  Data Store Memory20 : DataStoreMemory  DataStoreName=dTEstimnMagLLFil  StateMustResolveToSignalObject=on
  Data Store Memory21 : DataStoreMemory  DataStoreName=dTEstimnCuLLFil  StateMustResolveToSignalObject=on
  Data Store Memory22 : DataStoreMemory  DataStoreName=dTEstimnAssiMechLLFil  StateMustResolveToSignalObject=on
  Data Store Memory23 : DataStoreMemory  DataStoreName=dTEstimnWghtAvrgT  StateMustResolveToSignalObject=on
  Data Store Memory24 : DataStoreMemory  DataStoreName=AssiMechTInitEna  StateMustResolveToSignalObject=on
      settings: LockScale=on
  Data Store Memory26 : DataStoreMemory  DataStoreName=AmbTVldPrev  StateMustResolveToSignalObject=on
  Data Store Memory27 : DataStoreMemory  DataStoreName=EngOilTVldPrev  StateMustResolveToSignalObject=on
  Data Store Memory3 : DataStoreMemory  DataStoreName=MagTEstimnPrev  StateMustResolveToSignalObject=on
  Data Store Memory4 : DataStoreMemory  DataStoreName=CuFilLp  InitialValue=struct('FilSt',single(0),'FilGain',single(0))  OutDataTypeStr=Bus: FilLpRec1  StateMustResolveToSignalObject=on
  Data Store Memory5 : DataStoreMemory  DataStoreName=MagFilLp  InitialValue=struct('FilSt',single(0),'FilGain',single(0))  OutDataTypeStr=Bus: FilLpRec1  StateMustResolveToSignalObject=on
  Data Store Memory6 : DataStoreMemory  DataStoreName=AssiMechFilLp  InitialValue=struct('FilSt',single(0),'FilGain',single(0))  OutDataTypeStr=Bus: FilLpRec1  StateMustResolveToSignalObject=on
  Data Store Memory7 : DataStoreMemory  DataStoreName=CuTEstimnPrev  StateMustResolveToSignalObject=on
  Data Store Memory8 : DataStoreMemory  DataStoreName=SiFilLp  InitialValue=struct('FilSt',single(0),'FilGain',single(0))  OutDataTypeStr=Bus: FilLpRec1  StateMustResolveToSignalObject=on
  Data Store Memory9 : DataStoreMemory  DataStoreName=AssiMechTEstimnPrev  StateMustResolveToSignalObject=on
  Merge : Merge
  TEstimnInit1 : Subsystem  RequirementInfo={'linktype_rmi_doors' '0000a528 (/E-STEER Core/SubSystem Specifications/Application Functions/SF006A Temperature Estimation)' '#SF006A_143' 'true' 'REQ: SF006A_143' '' ; 'linktype_rmi_doors' '0000a528 (/E-STEER Core/SubSystem Specifications/Application Functions/SF006A Temperature Estimation)' '#SF006A_123' 'true' 'REQ: SF006A_123' '' } %GIDa_7c0d7579_f4de_4872_8bff_c0fcfba4d21b
  TEstimnPer1 : Subsystem  RequirementInfo={'linktype_rmi_doors' '0000a528 (/E-STEER Core/SubSystem Specifications/Application Functions/SF006A Temperature Estimation)' '#SF006A_173' 'true' 'REQ: SF006A_173' '' } %GIDa_804158cd_c0eb_4c52_b375_51081dcfcb4a
  MotFetT : Outport  RequirementInfo={'linktype_rmi_doors' '0000a528 (/E-STEER Core/SubSystem Specifications/Application Functions/SF006A Temperature Estimation)' '#SF006A_40' 'true' 'REQ: SF006A_40' '' } %GIDa_e043bfdf_9ab5_4c9d_accc_172393e56c12
  MotMagT : Outport  RequirementInfo={'linktype_rmi_doors' '0000a528 (/E-STEER Core/SubSystem Specifications/Application Functions/SF006A Temperature Estimation)' '#SF006A_41' 'true' 'REQ: SF006A_41' '' } %GIDa_6251f66c_4a70_4358_8419_9bbc744882ca  Port=2
  MotWidgT : Outport  RequirementInfo={'linktype_rmi_doors' '0000a528 (/E-STEER Core/SubSystem Specifications/Application Functions/SF006A Temperature Estimation)' '#SF006A_42' 'true' 'REQ: SF006A_42' '' } %GIDa_ad8986ff_f4d5_4df3_aeb3_1f00ee54b325  Port=3
  AssiMechT : Outport  RequirementInfo={'linktype_rmi_doors' '0000a528 (/E-STEER Core/SubSystem Specifications/Application Functions/SF006A Temperature Estimation)' '#SF006A_43' 'true' 'REQ: SF006A_43' '' } %GIDa_4d0d809e_eca0_4b44_a10e_3ac8781e6ac5  Port=4
  wires:
  call_TEstimnInit1/1 -> TEstimnInit1/Trigger
  AmbT/1 -> TEstimnPer1/1(AmbT), TEstimnInit1/1(AmbT)
  EcuTFild/1 -> TEstimnPer1/2(EcuTFild), TEstimnInit1/2(EcuTFild)
  EngOilT/1 -> TEstimnPer1/3(EngOilT), TEstimnInit1/3("EngOilT ")
  EngOilTVld/1 -> TEstimnPer1/4(EngOilTVld), TEstimnInit1/4("EngOilTVld ")
  AmbTVld/1 -> TEstimnPer1/5(AmbTVld), TEstimnInit1/5(AmbTVld)
  HwVel/1 -> TEstimnPer1/6(HwVel)
  MotCurrPeakEstimd/1 -> TEstimnPer1/7("MotCurrPeakEstimd ")
  AssiMechTEstimnDi/1 -> TEstimnPer1/8(AssiMechTEstimnDi)
  Bus Creator/1 -> Merge/1
  Bus Creator1/1 -> Merge/2
  Merge/1 -> Bus Selector/1
  call_TEstimnPer1/1 -> TEstimnPer1/Trigger
  Bus Selector/1 -> MotFetT/1  "<signal1>"
  Bus Selector/2 -> MotMagT/1  "<signal2>"
  Bus Selector/3 -> MotWidgT/1  "<signal3>"
  Bus Selector/4 -> AssiMechT/1  "<signal4>"
  TEstimnPer1/1(MotFetT) -> Bus Creator1/1
  TEstimnPer1/2(MotMagT) -> Bus Creator1/2
  TEstimnPer1/3(MotWidgT) -> Bus Creator1/3
  TEstimnPer1/4(AssiMechT) -> Bus Creator1/4
  TEstimnInit1/4(AssiMechT) -> Bus Creator/4
  TEstimnInit1/3(MotWidgT) -> Bus Creator/3
  TEstimnInit1/2(MotMagT) -> Bus Creator/2
  TEstimnInit1/1(MotFetT) -> Bus Creator/1

== system SF006A_TEstimn/call_TEstimnInit1 ==
  Enable : EnablePort
  Function-Call Generator : simulink/Ports & Subsystems/Function-Call Generator  sample_time=0  numberOfIterations=1
  Out1 : Outport
  wires:
  Function-Call Generator/1 -> Out1/1

== system SF006A_TEstimn/call_TEstimnPer1 ==
  Enable : EnablePort
  Function-Call Generator : simulink/Ports & Subsystems/Function-Call Generator  sample_time=0.1  numberOfIterations=1
  Out1 : Outport
  wires:
  Function-Call Generator/1 -> Out1/1

== system SF006A_TEstimn/TEstimn/Copyright1 ==

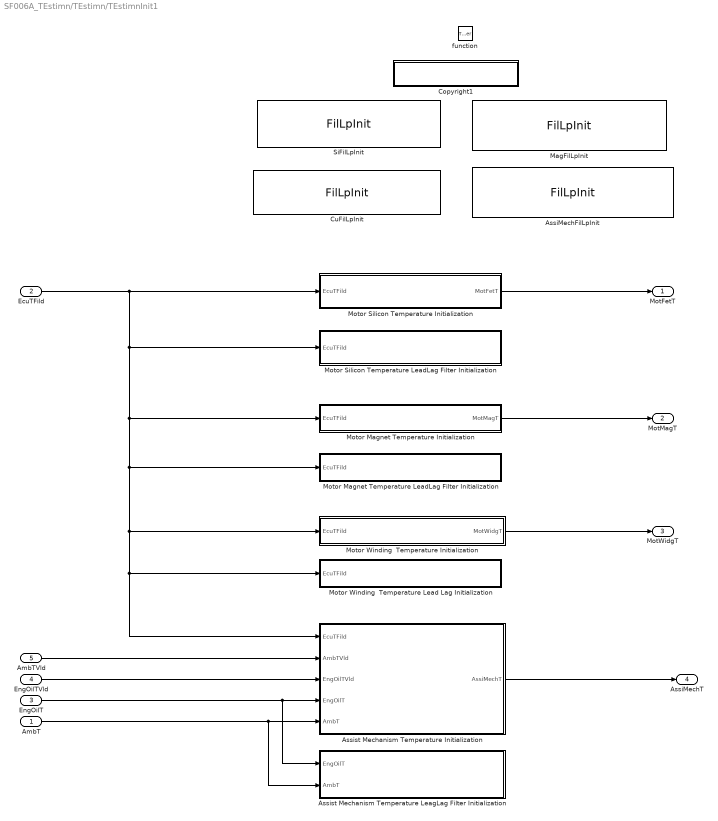
== system SF006A_TEstimn/TEstimn/TEstimnInit1 ==
  AmbT : Inport
  EcuTFild : Inport  Port=2
  "EngOilT " : Inport  Port=3
  "EngOilTVld " : Inport  Port=4
  AmbTVld : Inport  Port=5
  function : TriggerPort  TriggerType=function-call
  AssiMechFilLpInit : Fil/FilLpInit  Ic=0  Ts=ARCHGLBPRM_100MILLISEC_SEC_F32  Freq=TEstimnAssiMechAmbLpFilFrq  StVar=AssiMechFilLp
  Assist Mechanism Temperature Initialization : Subsystem
  Assist Mechanism Temperature LeagLag Filter Initialization : Subsystem
  Copyright1 : Subsystem  Description=|  RequirementInfo={} %GIDa_0a1cd7fa_88a7_493f_9ffa_3855db88fd16  mask(Copyright Information){none=on}
      | Copyright info block.                                               
      |                                                                     
      | Place copyright information at the top of every subsystem in design.
      mask prompts: none "No parameters"
      mask help: Place copyright information at the top of every subsystem in design.
      mask Display:
      | NxtrConf = 'Nexteer Confidential';
      | 
      | sys = bdroot; %handle for the current model ("system")
      | first = get_param(sys,'Created');
      | if(isempty(first))
      |     first = datestr(now,'yyyy');
      | else
      |     first = first(end-3:end);  %year is last four digits
      | end
      | 
      | last = get_param(sys,'LastModifiedDate');
      | if isempty(last)
      |     last = datestr(now,'yyyy');
      | else
      |     last = last(end-3:end);
      | end
      | 
      | if strcmp(first,last)
      |     fprintf('%s\nCopyright  %s Nexteer',NxtrConf,first);
      | else
      |     fprintf('%s\n%s%s-%s Nexteer',NxtrConf,char(169),first,last);
      | end
  CuFilLpInit : Fil/FilLpInit  Ic=0  Ts=ARCHGLBPRM_100MILLISEC_SEC_F32  Freq=TEstimnCuAmbLpFilFrq  StVar=CuFilLp
  MagFilLpInit : Fil/FilLpInit  Ic=0  Ts=ARCHGLBPRM_100MILLISEC_SEC_F32  Freq=TEstimnMagAmbLpFilFrq  StVar=MagFilLp
  Motor Magnet Temperature Initialization : Subsystem
  Motor Magnet Temperature LeadLag Filter Initialization : Subsystem  RequirementInfo={'linktype_rmi_doors' '0000a528 (/E-STEER Core/SubSystem Specifications/Application Functions/SF006A Temperature Estimation)' '#SF006A_171' 'true' 'REQ: SF006A_171' '' } %GIDa_19ccceac_e3b3_451e_aafd_5371ee054417
  Motor Silicon Temperature Initialization : Subsystem
  Motor Silicon Temperature LeadLag Filter Initialization : Subsystem  RequirementInfo={'linktype_rmi_doors' '0000a528 (/E-STEER Core/SubSystem Specifications/Application Functions/SF006A Temperature Estimation)' '#SF006A_171' 'true' 'REQ: SF006A_171' '' } %GIDa_01674f7c_7dcf_460a_add9_32f34e8d9998
  "Motor Winding  Temperature Initialization " : Subsystem
  "Motor Winding  Temperature Lead Lag Initialization " : Subsystem  RequirementInfo={'linktype_rmi_doors' '0000a528 (/E-STEER Core/SubSystem Specifications/Application Functions/SF006A Temperature Estimation)' '#SF006A_171' 'true' 'REQ: SF006A_171' '' } %GIDa_0847cd76_e7c5_422f_b0e5_90bd0dcbd6e6
  SiFilLpInit : Fil/FilLpInit  Ic=0  Ts=ARCHGLBPRM_100MILLISEC_SEC_F32  Freq=TEstimnSiAmbLpFilFrq  StVar=SiFilLp
  MotFetT : Outport
  MotMagT : Outport  Port=2
  MotWidgT : Outport  Port=3
  AssiMechT : Outport  Port=4
  wires:
  EcuTFild/1 -> Motor Silicon Temperature Initialization/1(EcuTFild), Motor Silicon Temperature LeadLag Filter Initialization/1(EcuTFild), Motor Magnet Temperature Initialization/1(EcuTFild), Motor Magnet Temperature LeadLag Filter Initialization/1(EcuTFild), "Motor Winding  Temperature Initialization "/1(EcuTFild), "Motor Winding  Temperature Lead Lag Initialization "/1(EcuTFild), Assist Mechanism Temperature Initialization/1(EcuTFild)
  Motor Silicon Temperature Initialization/1(MotFetT) -> MotFetT/1
  Motor Magnet Temperature Initialization/1(MotMagT) -> MotMagT/1
  "Motor Winding  Temperature Initialization "/1(MotWidgT) -> MotWidgT/1
  Assist Mechanism Temperature Initialization/1(AssiMechT) -> AssiMechT/1
  "EngOilT "/1 -> Assist Mechanism Temperature LeagLag Filter Initialization/1(EngOilT), Assist Mechanism Temperature Initialization/4("EngOilT ")
  AmbT/1 -> Assist Mechanism Temperature LeagLag Filter Initialization/2(AmbT), Assist Mechanism Temperature Initialization/5(AmbT)
  "EngOilTVld "/1 -> Assist Mechanism Temperature Initialization/3(EngOilTVld)
  AmbTVld/1 -> Assist Mechanism Temperature Initialization/2("AmbTVld ")

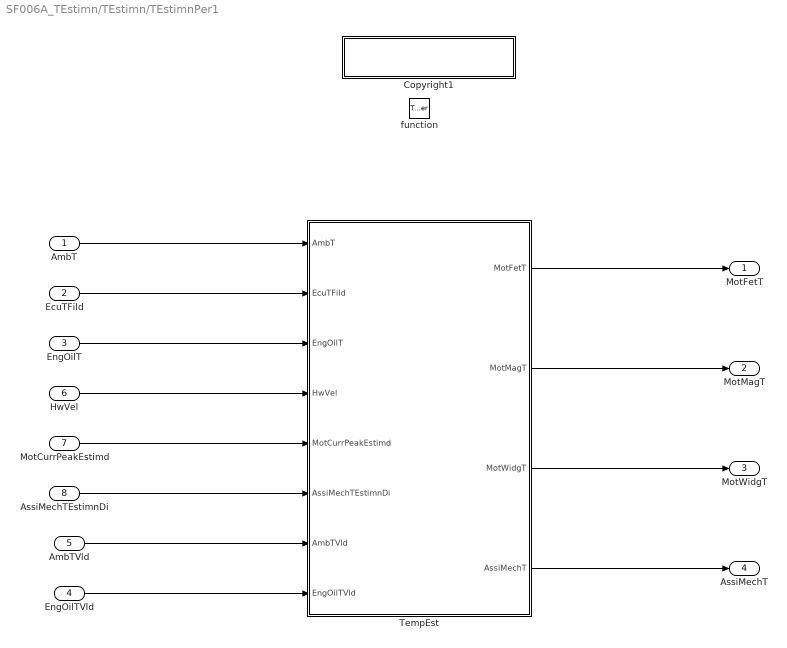
== system SF006A_TEstimn/TEstimn/TEstimnPer1 ==
  AmbT : Inport
  EcuTFild : Inport  Port=2
  EngOilT : Inport  Port=3
  EngOilTVld : Inport  Port=4
  AmbTVld : Inport  Port=5
  HwVel : Inport  Port=6
  "MotCurrPeakEstimd " : Inport  Port=7
  AssiMechTEstimnDi : Inport  Port=8
  function : TriggerPort  TriggerType=function-call
  Copyright1 : Subsystem  Description=|  RequirementInfo={} %GIDa_970fa5dd_e57d_4ad3_9415_7b101aee6356  mask(Copyright Information){none=on}
      | Copyright info block.                                               
      |                                                                     
      | Place copyright information at the top of every subsystem in design.
      mask prompts: none "No parameters"
      mask help: Place copyright information at the top of every subsystem in design.
      mask Display:
      | NxtrConf = 'Nexteer Confidential';
      | 
      | sys = bdroot; %handle for the current model ("system")
      | first = get_param(sys,'Created');
      | if(isempty(first))
      |     first = datestr(now,'yyyy');
      | else
      |     first = first(end-3:end);  %year is last four digits
      | end
      | 
      | last = get_param(sys,'LastModifiedDate');
      | if isempty(last)
      |     last = datestr(now,'yyyy');
      | else
      |     last = last(end-3:end);
      | end
      | 
      | if strcmp(first,last)
      |     fprintf('%s\nCopyright  %s Nexteer',NxtrConf,first);
      | else
      |     fprintf('%s\n%s%s-%s Nexteer',NxtrConf,char(169),first,last);
      | end
  TempEst : Subsystem  Tag=Temperature Estimation
      settings: AttributesFormatString=%<Tag>
  MotFetT : Outport
  MotMagT : Outport  Port=2
  MotWidgT : Outport  Port=3
  AssiMechT : Outport  Port=4
  wires:
  HwVel/1 -> TempEst/4("HwVel ")
  "MotCurrPeakEstimd "/1 -> TempEst/5("MotCurrPeakEstimd ")
  EngOilT/1 -> TempEst/3("EngOilT ")
  EcuTFild/1 -> TempEst/2(EcuTFild)
  AssiMechTEstimnDi/1 -> TempEst/6(AssiMechTEstimnDi)
  AmbT/1 -> TempEst/1("AmbT ")
  EngOilTVld/1 -> TempEst/8(EngOilTVld)
  AmbTVld/1 -> TempEst/7(AmbTVld)
  TempEst/4(AssiMechT) -> AssiMechT/1
  TempEst/3(MotWidgT) -> MotWidgT/1
  TempEst/2(MotMagT) -> MotMagT/1
  TempEst/1(MotFetT) -> MotFetT/1

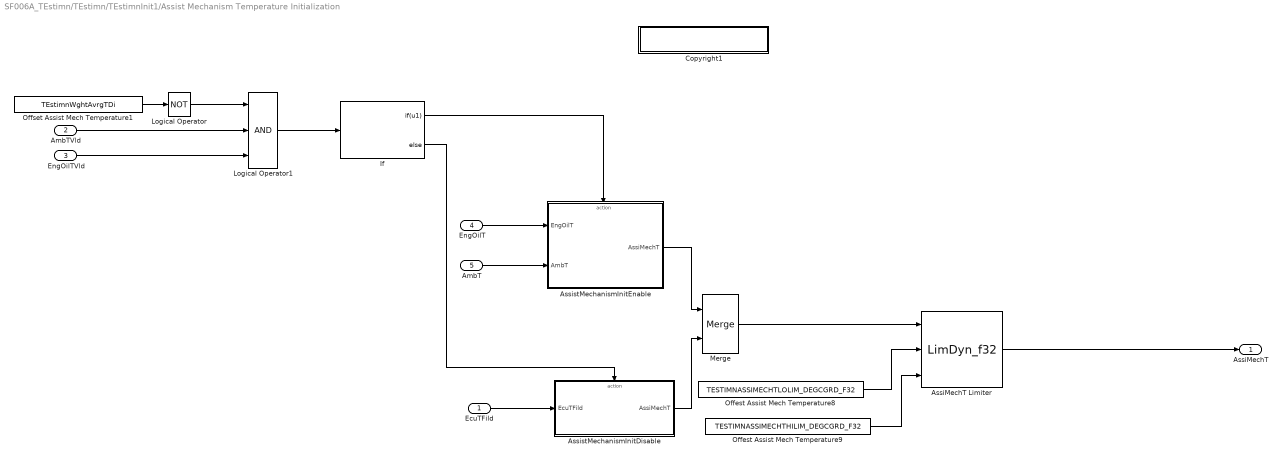
== system SF006A_TEstimn/TEstimn/TEstimnInit1/Assist Mechanism Temperature Initialization ==
  EcuTFild : Inport
  "AmbTVld " : Inport  Port=2
  EngOilTVld : Inport  RequirementInfo={} %GIDa_67dfbe45_b00e_437e_9e75_c022f6cb9cf0  Port=3
  "EngOilT " : Inport  Port=4
  AmbT : Inport  Port=5
  AssiMechT Limiter : NxtrLim/LimDyn_f32  RequirementInfo={'linktype_rmi_doors' '0000a528 (/E-STEER Core/SubSystem Specifications/Application Functions/SF006A Temperature Estimation)' '#SF006A_146' 'true' 'REQ: SF006A_146' '' } %GIDa_3e06bf1e_7cd0_4f39_a5b0_69df74191ecb
  AssistMechanismInitDisable : Subsystem
  AssistMechanismInitEnable : Subsystem
  Copyright1 : Subsystem  Description=|  RequirementInfo={} %GIDa_83985a7e_825b_4d63_a7b6_6f6e4cd34819  mask(Copyright Information){none=on}
      | Copyright info block.                                               
      |                                                                     
      | Place copyright information at the top of every subsystem in design.
      mask prompts: none "No parameters"
      mask help: Place copyright information at the top of every subsystem in design.
      mask Display:
      | NxtrConf = 'Nexteer Confidential';
      | 
      | sys = bdroot; %handle for the current model ("system")
      | first = get_param(sys,'Created');
      | if(isempty(first))
      |     first = datestr(now,'yyyy');
      | else
      |     first = first(end-3:end);  %year is last four digits
      | end
      | 
      | last = get_param(sys,'LastModifiedDate');
      | if isempty(last)
      |     last = datestr(now,'yyyy');
      | else
      |     last = last(end-3:end);
      | end
      | 
      | if strcmp(first,last)
      |     fprintf('%s\nCopyright  %s Nexteer',NxtrConf,first);
      | else
      |     fprintf('%s\n%s%s-%s Nexteer',NxtrConf,char(169),first,last);
      | end
  If : If  IfExpression=u1
  Logical Operator : Logic  Operator=NOT  AllPortsSameDT=off  OutDataTypeStr=boolean
  Logical Operator1 : Logic  Inputs=3  AllPortsSameDT=off  OutDataTypeStr=boolean
  Merge : Merge
  Offest Assist Mech Temperature8 : Constant  Value=TESTIMNASSIMECHTLOLIM_DEGCGRD_F32
  Offest Assist Mech Temperature9 : Constant  Value=TESTIMNASSIMECHTHILIM_DEGCGRD_F32
  Offset Assist Mech Temperature1 : Constant  Value=TEstimnWghtAvrgTDi
  AssiMechT : Outport
  wires:
  Logical Operator1/1 -> If/1
  "EngOilT "/1 -> AssistMechanismInitEnable/1("EngOilT ")
  AmbT/1 -> AssistMechanismInitEnable/2(AmbT)
  AssistMechanismInitEnable/1(AssiMechT) -> Merge/1
  If/1 -> AssistMechanismInitEnable/Action
  If/2 -> AssistMechanismInitDisable/Action
  EcuTFild/1 -> AssistMechanismInitDisable/1(EcuTFild)
  AssistMechanismInitDisable/1(AssiMechT) -> Merge/2
  Merge/1 -> AssiMechT Limiter/1
  Offest Assist Mech Temperature8/1 -> AssiMechT Limiter/2
  Offest Assist Mech Temperature9/1 -> AssiMechT Limiter/3
  AssiMechT Limiter/1 -> AssiMechT/1
  EngOilTVld/1 -> Logical Operator1/3
  "AmbTVld "/1 -> Logical Operator1/2
  Offset Assist Mech Temperature1/1 -> Logical Operator/1
  Logical Operator/1 -> Logical Operator1/1

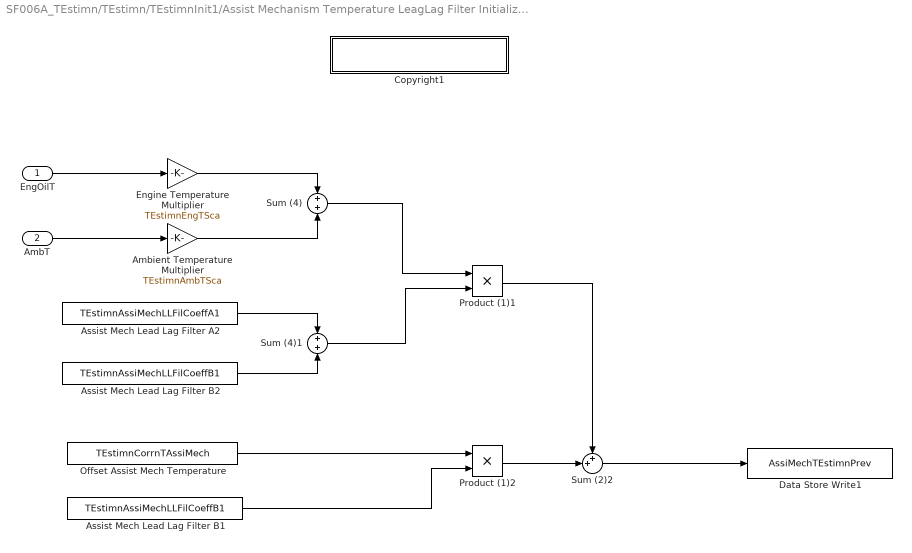
== system SF006A_TEstimn/TEstimn/TEstimnInit1/Assist Mechanism Temperature LeagLag Filter Initialization ==
  EngOilT : Inport
  AmbT : Inport  Port=2
  Ambient Temperature Multiplier : Gain  Gain=TEstimnAmbTSca
      settings: AttributesFormatString=%<Gain>
  Assist Mech Lead Lag Filter A2 : Constant  Value=TEstimnAssiMechLLFilCoeffA1
  Assist Mech Lead Lag Filter B1 : Constant  Value=TEstimnAssiMechLLFilCoeffB1
  Assist Mech Lead Lag Filter B2 : Constant  Value=TEstimnAssiMechLLFilCoeffB1
  Copyright1 : Subsystem  Description=|  RequirementInfo={} %GIDa_3105a6e9_84a8_4d8a_b6ed_34213f200397  mask(Copyright Information){none=on}
      | Copyright info block.                                               
      |                                                                     
      | Place copyright information at the top of every subsystem in design.
      mask prompts: none "No parameters"
      mask help: Place copyright information at the top of every subsystem in design.
      mask Display:
      | NxtrConf = 'Nexteer Confidential';
      | 
      | sys = bdroot; %handle for the current model ("system")
      | first = get_param(sys,'Created');
      | if(isempty(first))
      |     first = datestr(now,'yyyy');
      | else
      |     first = first(end-3:end);  %year is last four digits
      | end
      | 
      | last = get_param(sys,'LastModifiedDate');
      | if isempty(last)
      |     last = datestr(now,'yyyy');
      | else
      |     last = last(end-3:end);
      | end
      | 
      | if strcmp(first,last)
      |     fprintf('%s\nCopyright  %s Nexteer',NxtrConf,first);
      | else
      |     fprintf('%s\n%s%s-%s Nexteer',NxtrConf,char(169),first,last);
      | end
  Data Store Write1 : DataStoreWrite  DataStoreName=AssiMechTEstimnPrev
  Engine Temperature Multiplier : Gain  Gain=TEstimnEngTSca
      settings: AttributesFormatString=%<Gain>
  Offset Assist Mech Temperature : Constant  Value=TEstimnCorrnTAssiMech
  Product (1)1 : Product  RndMeth=Zero
  Product (1)2 : Product  RndMeth=Zero
  Sum (2)2 : Sum  Inputs=++|
  Sum (4) : Sum  Inputs=+|+
  Sum (4)1 : Sum  Inputs=+|+
  wires:
  EngOilT/1 -> Engine Temperature Multiplier/1
  Engine Temperature Multiplier/1 -> Sum (4)/1
  Ambient Temperature Multiplier/1 -> Sum (4)/2
  AmbT/1 -> Ambient Temperature Multiplier/1
  Sum (4)/1 -> Product (1)1/1
  Sum (4)1/1 -> Product (1)1/2
  Assist Mech Lead Lag Filter A2/1 -> Sum (4)1/1
  Assist Mech Lead Lag Filter B2/1 -> Sum (4)1/2
  Offset Assist Mech Temperature/1 -> Product (1)2/1
  Assist Mech Lead Lag Filter B1/1 -> Product (1)2/2
  Product (1)1/1 -> Sum (2)2/1
  Product (1)2/1 -> Sum (2)2/2
  Sum (2)2/1 -> Data Store Write1/1

== system SF006A_TEstimn/TEstimn/TEstimnInit1/Copyright1 ==

== system SF006A_TEstimn/TEstimn/TEstimnInit1/Motor Magnet Temperature Initialization ==
  EcuTFild : Inport
  Copyright1 : Subsystem  Description=|  RequirementInfo={} %GIDa_d4777a6c_99a5_4474_b89d_de3e9ab965fb  mask(Copyright Information){none=on}
      | Copyright info block.                                               
      |                                                                     
      | Place copyright information at the top of every subsystem in design.
      mask prompts: none "No parameters"
      mask help: Place copyright information at the top of every subsystem in design.
      mask Display:
      | NxtrConf = 'Nexteer Confidential';
      | 
      | sys = bdroot; %handle for the current model ("system")
      | first = get_param(sys,'Created');
      | if(isempty(first))
      |     first = datestr(now,'yyyy');
      | else
      |     first = first(end-3:end);  %year is last four digits
      | end
      | 
      | last = get_param(sys,'LastModifiedDate');
      | if isempty(last)
      |     last = datestr(now,'yyyy');
      | else
      |     last = last(end-3:end);
      | end
      | 
      | if strcmp(first,last)
      |     fprintf('%s\nCopyright  %s Nexteer',NxtrConf,first);
      | else
      |     fprintf('%s\n%s%s-%s Nexteer',NxtrConf,char(169),first,last);
      | end
  MotMagT Limiter : NxtrLim/LimDyn_f32  RequirementInfo={'linktype_rmi_doors' '0000a528 (/E-STEER Core/SubSystem Specifications/Application Functions/SF006A Temperature Estimation)' '#SF006A_145' 'true' 'REQ: SF006A_145' '' ; 'linktype_rmi_doors' '0000a528 (/E-STEER Core/SubSystem Specifications/Application Functions/SF006A Temperature Estimation)' '#SF006A_147' 'true' 'REQ: SF006A_147' '' } %GIDa_701b9a22_13d0_444d_956f_26edba067845
  Offest Assist Mech Temperature4 : Constant  Value=TESTIMNMAGTLOLIM_DEGCGRD_F32
  Offest Assist Mech Temperature5 : Constant  Value=TESTIMNMAGTHILIM_DEGCGRD_F32
  MotMagT : Outport
  wires:
  MotMagT Limiter/1 -> MotMagT/1
  Offest Assist Mech Temperature5/1 -> MotMagT Limiter/3
  EcuTFild/1 -> MotMagT Limiter/1
  Offest Assist Mech Temperature4/1 -> MotMagT Limiter/2

== system SF006A_TEstimn/TEstimn/TEstimnInit1/Motor Magnet Temperature LeadLag Filter Initialization ==
  EcuTFild : Inport
  Copyright1 : Subsystem  Description=|  RequirementInfo={} %GIDa_09c0424e_2a25_4a5a_adc2_6f7be29435eb  mask(Copyright Information){none=on}
      | Copyright info block.                                               
      |                                                                     
      | Place copyright information at the top of every subsystem in design.
      mask prompts: none "No parameters"
      mask help: Place copyright information at the top of every subsystem in design.
      mask Display:
      | NxtrConf = 'Nexteer Confidential';
      | 
      | sys = bdroot; %handle for the current model ("system")
      | first = get_param(sys,'Created');
      | if(isempty(first))
      |     first = datestr(now,'yyyy');
      | else
      |     first = first(end-3:end);  %year is last four digits
      | end
      | 
      | last = get_param(sys,'LastModifiedDate');
      | if isempty(last)
      |     last = datestr(now,'yyyy');
      | else
      |     last = last(end-3:end);
      | end
      | 
      | if strcmp(first,last)
      |     fprintf('%s\nCopyright  %s Nexteer',NxtrConf,first);
      | else
      |     fprintf('%s\n%s%s-%s Nexteer',NxtrConf,char(169),first,last);
      | end
  Data Store Write1 : DataStoreWrite  DataStoreName=MagTEstimnPrev
  Magnet Lead Lag Filter A1 : Constant  Value=TEstimnMagLLFilCoeffA1
  Magnet Lead Lag Filter B1 : Constant  Value=TEstimnMagLLFilCoeffB1
  Offset Copper Temperature1 : Constant  Value=TEstimnCorrnTMag
  Product (1) : Product  RndMeth=Zero
  Product (2) : Product  RndMeth=Zero
  Product (3) : Product  RndMeth=Zero
  Sum (2) : Sum  Inputs=++|
  Sum (2)1 : Sum  Inputs=++|
  wires:
  Magnet Lead Lag Filter A1/1 -> Product (3)/2
  Product (2)/1 -> Sum (2)1/1
  Magnet Lead Lag Filter B1/1 -> Product (1)/2, Product (2)/1
  Product (1)/1 -> Sum (2)/1
  Sum (2)/1 -> Data Store Write1/1
  Sum (2)1/1 -> Sum (2)/2
  Product (3)/1 -> Sum (2)1/2
  EcuTFild/1 -> Product (3)/1, Product (2)/2
  Offset Copper Temperature1/1 -> Product (1)/1

== system SF006A_TEstimn/TEstimn/TEstimnInit1/Motor Silicon Temperature Initialization ==
  EcuTFild : Inport
  Copyright1 : Subsystem  Description=|  RequirementInfo={} %GIDa_43cb6b3a_c460_44f6_9088_0cf9d127a797  mask(Copyright Information){none=on}
      | Copyright info block.                                               
      |                                                                     
      | Place copyright information at the top of every subsystem in design.
      mask prompts: none "No parameters"
      mask help: Place copyright information at the top of every subsystem in design.
      mask Display:
      | NxtrConf = 'Nexteer Confidential';
      | 
      | sys = bdroot; %handle for the current model ("system")
      | first = get_param(sys,'Created');
      | if(isempty(first))
      |     first = datestr(now,'yyyy');
      | else
      |     first = first(end-3:end);  %year is last four digits
      | end
      | 
      | last = get_param(sys,'LastModifiedDate');
      | if isempty(last)
      |     last = datestr(now,'yyyy');
      | else
      |     last = last(end-3:end);
      | end
      | 
      | if strcmp(first,last)
      |     fprintf('%s\nCopyright  %s Nexteer',NxtrConf,first);
      | else
      |     fprintf('%s\n%s%s-%s Nexteer',NxtrConf,char(169),first,last);
      | end
  MotFetT Limiter : NxtrLim/LimDyn_f32  RequirementInfo={'linktype_rmi_doors' '0000a528 (/E-STEER Core/SubSystem Specifications/Application Functions/SF006A Temperature Estimation)' '#SF006A_145' 'true' 'REQ: SF006A_145' '' ; 'linktype_rmi_doors' '0000a528 (/E-STEER Core/SubSystem Specifications/Application Functions/SF006A Temperature Estimation)' '#SF006A_147' 'true' 'REQ: SF006A_147' '' } %GIDa_4d2942e9_1947_44cb_8ccb_eb841246889e
  Offest Assist Mech Temperature2 : Constant  Value=TESTIMNFETTLOLIM_DEGCGRD_F32
  Offest Assist Mech Temperature3 : Constant  Value=TESTIMNFETTHILIM_DEGCGRD_F32
  MotFetT : Outport
  wires:
  Offest Assist Mech Temperature3/1 -> MotFetT Limiter/3
  EcuTFild/1 -> MotFetT Limiter/1
  Offest Assist Mech Temperature2/1 -> MotFetT Limiter/2
  MotFetT Limiter/1 -> MotFetT/1

== system SF006A_TEstimn/TEstimn/TEstimnInit1/Motor Silicon Temperature LeadLag Filter Initialization ==
  EcuTFild : Inport
  Copyright1 : Subsystem  Description=|  RequirementInfo={} %GIDa_988db9eb_4f24_4678_a531_5a26a31603e2  mask(Copyright Information){none=on}
      | Copyright info block.                                               
      |                                                                     
      | Place copyright information at the top of every subsystem in design.
      mask prompts: none "No parameters"
      mask help: Place copyright information at the top of every subsystem in design.
      mask Display:
      | NxtrConf = 'Nexteer Confidential';
      | 
      | sys = bdroot; %handle for the current model ("system")
      | first = get_param(sys,'Created');
      | if(isempty(first))
      |     first = datestr(now,'yyyy');
      | else
      |     first = first(end-3:end);  %year is last four digits
      | end
      | 
      | last = get_param(sys,'LastModifiedDate');
      | if isempty(last)
      |     last = datestr(now,'yyyy');
      | else
      |     last = last(end-3:end);
      | end
      | 
      | if strcmp(first,last)
      |     fprintf('%s\nCopyright  %s Nexteer',NxtrConf,first);
      | else
      |     fprintf('%s\n%s%s-%s Nexteer',NxtrConf,char(169),first,last);
      | end
  Data Store Write1 : DataStoreWrite  DataStoreName=SiTEstimnPrev
  Offset Copper Temperature : Constant  Value=TEstimnCorrnTSi
  Product (1) : Product  RndMeth=Zero
  Product (2) : Product  RndMeth=Zero
  Product (3) : Product  RndMeth=Zero
  Silicon Lead Lag Filter A1 : Constant  Value=TEstimnSiLLFilCoeffA1
  Silicon Lead Lag Filter B1 : Constant  Value=TEstimnSiLLFilCoeffB1
  Sum (2) : Sum  Inputs=++|
  Sum (2)1 : Sum  Inputs=++|
  wires:
  Silicon Lead Lag Filter A1/1 -> Product (3)/2
  Silicon Lead Lag Filter B1/1 -> Product (1)/2, Product (2)/1
  Sum (2)1/1 -> Data Store Write1/1
  Product (1)/1 -> Sum (2)1/1
  Product (3)/1 -> Sum (2)/2
  Sum (2)/1 -> Sum (2)1/2
  EcuTFild/1 -> Product (2)/2, Product (3)/1
  Offset Copper Temperature/1 -> Product (1)/1
  Product (2)/1 -> Sum (2)/1

== system SF006A_TEstimn/TEstimn/TEstimnInit1/Motor Winding  Temperature Initialization  ==
  EcuTFild : Inport
  Copyright1 : Subsystem  Description=|  RequirementInfo={} %GIDa_5709b085_f9d1_464a_b4eb_6d79c1137d28  mask(Copyright Information){none=on}
      | Copyright info block.                                               
      |                                                                     
      | Place copyright information at the top of every subsystem in design.
      mask prompts: none "No parameters"
      mask help: Place copyright information at the top of every subsystem in design.
      mask Display:
      | NxtrConf = 'Nexteer Confidential';
      | 
      | sys = bdroot; %handle for the current model ("system")
      | first = get_param(sys,'Created');
      | if(isempty(first))
      |     first = datestr(now,'yyyy');
      | else
      |     first = first(end-3:end);  %year is last four digits
      | end
      | 
      | last = get_param(sys,'LastModifiedDate');
      | if isempty(last)
      |     last = datestr(now,'yyyy');
      | else
      |     last = last(end-3:end);
      | end
      | 
      | if strcmp(first,last)
      |     fprintf('%s\nCopyright  %s Nexteer',NxtrConf,first);
      | else
      |     fprintf('%s\n%s%s-%s Nexteer',NxtrConf,char(169),first,last);
      | end
  MotWidgT Limiter : NxtrLim/LimDyn_f32  RequirementInfo={'linktype_rmi_doors' '0000a528 (/E-STEER Core/SubSystem Specifications/Application Functions/SF006A Temperature Estimation)' '#SF006A_145' 'true' 'REQ: SF006A_145' '' ; 'linktype_rmi_doors' '0000a528 (/E-STEER Core/SubSystem Specifications/Application Functions/SF006A Temperature Estimation)' '#SF006A_147' 'true' 'REQ: SF006A_147' '' } %GIDa_66d33ade_9142_4d58_ba23_def66d59f0c0
  Offest Assist Mech Temperature6 : Constant  Value=TESTIMNWIDGTLOLIM_DEGCGRD_F32
  Offest Assist Mech Temperature7 : Constant  Value=TESTIMNWIDGTHILIM_DEGCGRD_F32
  MotWidgT : Outport
  wires:
  Offest Assist Mech Temperature7/1 -> MotWidgT Limiter/3
  EcuTFild/1 -> MotWidgT Limiter/1
  Offest Assist Mech Temperature6/1 -> MotWidgT Limiter/2
  MotWidgT Limiter/1 -> MotWidgT/1

== system SF006A_TEstimn/TEstimn/TEstimnInit1/Motor Winding  Temperature Lead Lag Initialization  ==
  EcuTFild : Inport
  Copper Lead Lag Filter A1 : Constant  Value=TEstimnCuLLFilCoeffA1
  Copper Lead Lag Filter B1 : Constant  Value=TEstimnCuLLFilCoeffB1
  Copyright1 : Subsystem  Description=|  RequirementInfo={} %GIDa_41aacf8b_4c51_4fbb_b0d4_b62ce1c2d424  mask(Copyright Information){none=on}
      | Copyright info block.                                               
      |                                                                     
      | Place copyright information at the top of every subsystem in design.
      mask prompts: none "No parameters"
      mask help: Place copyright information at the top of every subsystem in design.
      mask Display:
      | NxtrConf = 'Nexteer Confidential';
      | 
      | sys = bdroot; %handle for the current model ("system")
      | first = get_param(sys,'Created');
      | if(isempty(first))
      |     first = datestr(now,'yyyy');
      | else
      |     first = first(end-3:end);  %year is last four digits
      | end
      | 
      | last = get_param(sys,'LastModifiedDate');
      | if isempty(last)
      |     last = datestr(now,'yyyy');
      | else
      |     last = last(end-3:end);
      | end
      | 
      | if strcmp(first,last)
      |     fprintf('%s\nCopyright  %s Nexteer',NxtrConf,first);
      | else
      |     fprintf('%s\n%s%s-%s Nexteer',NxtrConf,char(169),first,last);
      | end
  Data Store Write1 : DataStoreWrite  DataStoreName=CuTEstimnPrev
  Offset Copper Temperature : Constant  Value=TEstimnCorrnTCu
  Product (1) : Product  RndMeth=Zero
  Product (2) : Product  RndMeth=Zero
  Product (3) : Product  RndMeth=Zero
  Sum (2) : Sum  Inputs=++|
  Sum (3)1 : Sum  Inputs=++|
  wires:
  Copper Lead Lag Filter A1/1 -> Product (3)/2
  Copper Lead Lag Filter B1/1 -> Product (1)/2, Product (2)/1
  Product (1)/1 -> Sum (2)/1
  Sum (2)/1 -> Data Store Write1/1
  EcuTFild/1 -> Product (2)/2, Product (3)/1
  Offset Copper Temperature/1 -> Product (1)/1
  Product (3)/1 -> Sum (3)1/2
  Product (2)/1 -> Sum (3)1/1
  Sum (3)1/1 -> Sum (2)/2

== system SF006A_TEstimn/TEstimn/TEstimnPer1/Copyright1 ==
